simulink library "AEMS_Standard_Library"  (R2016b)
(part 4 of 39)

      |             end
      |         end
      |     end
      | 
      | %% Delete all AEMS_FLOAT_TO_FXP_WITH_LIMIT and AEMS_EXTRACT_BIT blocks
      |     k2=[find_system(hh,'FollowLinks','on','LookunderMasks','all','regexp','on','Name','^AEMS_TO_FXP_WITH_LIMIT');find_system(hh,'FollowLinks','on','LookunderMasks','all','MaskType','AEMS_EXTRACT_BIT')];
      | % if size(k,1)~= str2num(buf)
      |     for j = 1:length(k2)
      |         try
      |             delete_block(k2{j});
      |         end
      |     end
      | 
      | %% Settings for the Mux
      | % Number of inputs
      |     set_param([hh '/Mux'],'Inputs',num2str(buff_size));
      | 
      | % Mux position
      |     Blk.Position=get_param([hh '/Mux'],'position');
      |     Position = Blk.Position;
      |     Position(2) = pos(2) - 60*buff_size;
      |     Position(4) = pos(2) + 60*buff_size;
      |     set_param([hh '/Mux'],'Position', Position);
      |     inblkhandles=get_param([hh '/Mux'], 'PortHandles');
      | 
      |     set_param(hh,'Position',conv_sub_pos);
      | %% For each DID, recreate it
      |     i=0;
      |     txtvisibility='%<MaskType> \n DID Abstract: %<DIDAbstract> \n Number of DID Variables: %<NumDIDVar> ';
      |     for k=1:countDID
      |         k_str = num2str(k);
      | 
      |       try
      |         %% Add the DID information into the displayed text under the main lib block
      |         txtvisibility=[txtvisibility,'\n %<In_DID_Name_',k_str,'> : {','Range = %<RaDIDVar',k_str,'>, Resol = %<ResolDIDVar',k_str,'>, Offset = %<OffsetDIDVar',k_str,'>, DID Data Type= %<DataTypeDIDVar',k_str,'>}'];
      |         
      |         %% Retrieve all data from the DID tab  
      |         tRange = strsplit(strrep(strrep(strrep(get_param(libcb,['RaDIDVar',k_str]),' ',''),'[',''),']',''),',');
      |         tMin = tRange{1};
      |         tMax = tRange{2}; 
      |         tResol = get_param(libcb,['ResolDIDVar',k_str]);
      |         tOffset = get_param(libcb,['OffsetDIDVar',k_str]);
      |         
      |         tByte = get_param(libcb,['DataTypeDIDVar',k_str]);
      |         if(strcmp(tByte, 'int8') || strcmp (tByte, 'uint8'))
      |             t_buff_size=1;
      |         elseif(strcmp(tByte, 'int16') || strcmp (tByte, 'uint16'))
      |             t_buff_size=2;
      |         else
      |             t_buff_size=4;
      |         end
      |         
      | %% For each element in the buffer
      |         for ii=1:t_buff_size
      |             i=i+1;
      |             i_str = num2str(i);
      |             pos=get_param(inblkhandles.Inport(i),'position');
      |             cur_ext_bit = [hh '/AEMS_EXTRACT_BIT_',i_str];
      | 
      | %% Adding AEMS_EXTRACT_BIT if buffer > 1
      | % Adding block 
      |             if t_buff_size >= 1
      |                 add_block('AEMS_Standard_Library/BIT_OPERATION/AEMS_EXTRACT_BIT',cur_ext_bit,'Position',[pos(1)-300 pos(2)-15 pos(1)-100 pos(2)+15]);
      |                 %                     add_block('AEMS_Standard_Library/BIT_OPERATION/AEMS_EXTRACT_BIT',[hh '/AEMS_EXTRACT_BIT_' num2str(i)],'Position',[pos(1)-320 pos(2)-25 pos(1)-140 pos(2)+25]);
      |                 set_param(cur_ext_bit,'Value','Range of bits');
      |                 set_param(cur_ext_bit,'DataType',tByte);
      |             end
      |             
      | %% For the first byte in the buffer only, we create the input and float and fxp
      |             if ii==1
      |                 name_inpo = get_param(libcb,['In_DID_Name_',k_str]);
      |                 try
      |                     add_block('built-in/Inport',[hh '/DID_Variable_',k_str],'Position',[140 pos(2)-6 160 pos(2)+6],'BackGroundColor','Green');
      |                 catch
      |                   set_param([hh '/DID_Variable_',k_str],'Position',[140 pos(2)-6 160 pos(2)+6]);
      |                 end
      |                 
      | %% Add DataTypeConversion or AEMS_FLOAT_TO_FXP_WITH_LIMIT, and name them AEMS_FLOAT_TO_FXP_WITH_LIMIT_XX
      | % Remark Etienne: Not sure this part is right. User expects his data to be maxed at 1 in this case.               
      |                 flag_convert = 0;
      |                 try
      |                     if isequal({tResol,tMin,tMax,tOffset,tByte},{'1','0','1','0','1'})
      |                         add_block('built-in/DataTypeConversion',[hh '/AEMS_TO_FXP_WITH_LIMIT_',k_str],'Position',[pos(1)-620 pos(2)-20 pos(1)-555 pos(2)+15],'ShowName','off');
      |                         flag_convert = 1;
      |                     else
      |                         add_block('AEMS_Standard_Library/DCM/AEMS_TO_FXP_WITH_LIMIT',[hh '/AEMS_TO_FXP_WITH_LIMIT_',k_str],'Position',[pos(1)-720 pos(2)-20 pos(1)-460 pos(2)+20]);
      |                         set_param([hh '/AEMS_TO_FXP_WITH_LIMIT_',k_str],'OutputFixedPointDatatype',tByte);%Data type has to be set first before setting other attributes.                        
      |                         set_param([hh '/AEMS_TO_FXP_WITH_LIMIT_',k_str],...
      |                             'Resol',tResol,...
      |                             'Min',tMin,...
      |                             'Max',tMax,...
      |                             'Offset',tOffset);
      |                     end
      |                 end
      |                 
      | %% Setting lines and adding the inport
      |                 inp_k_pos = [40 conv_sub_pos(2)+10 60 conv_sub_pos(2)+22];
      |                 try
      |                     %                             add_line(hh,[name_inpo,'/1'],['AEMS_TO_FXP_WITH_LIMIT_',k_str,'/1'],'Autorouting','On');
      |                     
      |                     add_line(hh,['DID_Variable_',k_str,'/1'],['AEMS_TO_FXP_WITH_LIMIT_',k_str,'/1'],'Autorouting','On');
      |                     %                         add_block('built-in/Inport',[libcb '/DID_Variable_' num2str(k)],'Position',[posport(1)-10 posport(2)-6+k*100 posport(1)+10 posport(2)+6+k*100],'BackGroundColor','Green');
      |                     add_block('built-in/Inport',[libcb,'/DID_Variable_',k_str],'Position',inp_k_pos,'BackGroundColor','Green');
      |                     add_line(libcb,['DID_Variable_',k_str,'/1'],['Conversion_Subsystem/',k_str],'Autorouting','On');
      |                 catch
      |                     %                                                     set_param([libcb '/DID_Variable_' num2str(k)],'Position',[posport(1)-10 posport(2)-6+k*100 posport(1)+10 posport(2)+6+k*100]);
      |                     set_param([libcb,'/DID_Variable_',k_str],'Position',inp_k_pos);
      |                 end
      |             end
      |             
      |  %% Setting the range of bits to extract
      |             Start_Bit = (t_buff_size-ii)*8;
      |             End_Bit   = Start_Bit + 7;
      |             Range_Of_Bits = ['[',num2str(Start_Bit),',',num2str(End_Bit),']'];
      |             set_param(cur_ext_bit,'Range',Range_Of_Bits);
      |             
      | %% Linking the AEMS_FLOAT_TO_FXP_WITH_LIMIT and AEMS_EXTRACT_BIT_
      |             if t_buff_size > 0
      |                 add_line(hh,['AEMS_TO_FXP_WITH_LIMIT_',k_str,'/1'],['AEMS_EXTRACT_BIT_' num2str(i),'/1'], 'Autorouting','On');
      |                 add_line(hh,['AEMS_EXTRACT_BIT_',i_str,'/1'],['Mux/',i_str], 'Autorouting','On');
      |             end
      |         end
      |         
      |     catch error
      |         disp(error.message);
      |     end
      | end
      | 
      | %% Linking the inport for the Conversion_Subsystem
      |     ph_hh = get_param(hh,'PortHandles');
      |     ph_hh_in = ph_hh.Inport;
      |     for k1 = 1:countDID
      |         k1_str = num2str(k1);
      |         ph_hh_in_pos = get(ph_hh_in(k1),'Position');
      |         inp_k_pos = [40 ph_hh_in_pos(2)-6 60 ph_hh_in_pos(2)+6];
      |         set_param([libcb,'/DID_Variable_',k1_str],'Position',inp_k_pos);
      |         %             set_param([libcb,'/',name_inp1],'Position',inp_k_pos);
      |         try
      |             delete_line(libcb,['DID_Variable_',k1_str,'/1'],['Conversion_Subsystem/',k1_str]);
      |         catch
      |             disp('sf');
      |         end
      |         add_line(libcb,['DID_Variable_',k1_str,'/1'],['Conversion_Subsystem/',k1_str],'Autorouting','On');
      |     end
      |     
      | %% Setting position of the block relatively to the number of inputs
      |     prs_pos = get_param(libcb,'Position');
      |     if countDID > 4
      |         set_param(libcb,'Position',[prs_pos(1) prs_pos(2) prs_pos(3) prs_pos(2)+(countDID*30)]);
      |     else
      |         set_param(libcb,'Position',[prs_pos(1) prs_pos(2) prs_pos(3) prs_pos(2)+120]);
      |     end
      |     set_param(libcb,'AttributesFormatString',txtvisibility);
      | end
      | %% Setting the name of the DID in the inports
      |     fin_ip = find_system(libh,'LookUnderMasks','all','FollowLinks','on','SearchDepth','1','BlockType','Inport');
      |     for ip_cnt=1:length(fin_ip)
      |      cur_ip_name = get_param(libcb,['In_DID_Name_',num2str(ip_cnt)]);
      |         if ~isnan(str2double(cur_ip_name)) && isnumeric(str2double(cur_ip_name))
      |          errordlg(['invalid inport name entered for DID variable',num2str(ip_cnt)]);
      |         elseif ~isempty(cur_ip_name)
      |         try
      |             set(fin_ip(ip_cnt),'Name',cur_ip_name);
      |         catch
      |             errordlg(['invalid/duplicate inport name entered for DID variable',num2str(ip_cnt)]);
      |         end
      |         end
      |     end
      settings: AttributesFormatString=%<MaskType> \n DID Abstract: %<DIDAbstract> \n Number of DID Variables: %<NumDIDVar> \n %<In_DID_Name_1> : {Range = %<RaDIDVar1>, Resol = %<ResolDIDVar1>, Offset = %<OffsetDIDVar1>, DID Data Type= %<DataTypeDIDVar1>}
      mask Help:
      | eval('path_lib=fileparts(which(''AEMS_Standard_Library''));');
      | doc_path = [path_lib '\help\AEMS_DCM_DID_READDATA.pdf'];
      | eval('open(doc_path)')
      mask TypeOptions NumDIDVar: 1 | 2 | 3 | 4 | 5 | 6 | 7 | 8 | 9 | 10 | 11 | 12 | 13 | 14 | 15 | 16 | 17 | 18 | 19 | 20 | 21 | 22 | 23 | 24 | 25 | 26 | 27 | 28 | 29 | 30 | 31 | 32 | 33 | 34 | 35 | 36 | 37 | 38 | 39 | 40 | 41 | 42 | 43 | 44 | 45 | 46 | 47 | 48 | 49 | 50 | 51 | 52 | 53 | 54 | 55 | 56 | 57 | 58 | 59 | 60 | 61 | 62 | 63 | 64 | 65 | 66 | 67 | 68 | 69 | 70 | 71 | 72 | 73 | 74 | 75 | 76 | 77 | 78 | 79 | 80 | 81 | 82 | 83 | 84 | 85 | 86 | 87 | 88 | 89 | 90 | 91 | 92 | 93 | 94 | 95 | 96 | 97 | 98 | 99 | 100 | 101 | 102 | 103 | 104 | 105 | 106 | 107 | 108 | 109 | 110 | 111 | 112 | 113 | 114 | 115 | 116 | 117 | 118 | 119 | 120 | 121 | 122 | 123 | 124 | 125 | 126 | 127 | 128 | 129 | 130 | 131 | 132 | 133 | 134 | 135 | 136 | 137 | 138 | 139 | 140 | 141 | 142 | 143 | 144 | 145 | 146 | 147 | 148 | 149 | 150 | 151 | 152 | 153 | 154 | 155 | 156 | 157 | 158 | 159 | 160 | 161 | 162 | 163 | 164 | 165 | 166 | 167 | 168 | 169 | 170 | 171 | 172 | 173 | 174 | 175 | 176 | 177 | 178 | 179 | 180 | 181 | 182 | 183 | 184 | 185 | 186 | 187 | 188 | 189 | 190 | 191 | 192 | 193 | 194 | 195 | 196 | 197 | 198 | 199 | 200 | 201 | 202 | 203 | 204 | 205 | 206 | 207 | 208 | 209 | 210 | 211 | 212 | 213 | 214 | 215 | 216 | 217 | 218 | 219 | 220 | 221 | 222 | 223 | 224 | 225 | 226 | 227 | 228 | 229 | 230 | 231 | 232 | 233 | 234 | 235 | 236 | 237 | 238 | 239 | 240 | 241 | 242 | 243 | 244 | 245 | 246 | 247 | 248 | 249 | 250 | 251 | 252 | 253 | 254 | 255 | 256 | 257 | 258 | 259 | 260 | 261 | 262 | 263 | 264 | 265 | 266 | 267 | 268 | 269 | 270 | 271 | 272 | 273 | 274 | 275 | 276 | 277 | 278 | 279 | 280 | 281 | 282 | 283 | 284 | 285 | 286 | 287 | 288 | 289 | 290 | 291 | 292 | 293 | 294 | 295 | 296 | 297 | 298 | 299 | 300 | 301 | 302 | 303 | 304 | 305 | 306 | 307 | 308 | 309 | 310 | 311 | 312 | 313 | 314 | 315 | 316 | 317 | 318 | 319 | 320 | 321 | 322 | 323 | 324 | 325 | 326 | 327 | 328 | 329 | 330 | 331 | 332 | 333 | 334 | 335 | 336 | 337 | 338 | 339 | 340 | 341 | 342 | 343 | 344 | 345 | 346 | 347 | 348 | 349 | 350 | 351 | 352 | 353 | 354 | 355 | 356 | 357 | 358 | 359 | 360 | 361 | 362 | 363 | 364 | 365 | 366 | 367 | 368 | 369 | 370 | 371 | 372 | 373 | 374 | 375 | 376 | 377 | 378 | 379 | 380 | 381 | 382 | 383 | 384 | 385 | 386 | 387 | 388 | 389 | 390 | 391 | 392 | 393 | 394 | 395 | 396 | 397 | 398 | 399 | 400
      mask Callback NumDIDVar:
      | mo = get_param(gcb,'MaskObject');
      | %Get number of tabs in container 2
      | NumOfTabs = mo.getDialogControl('tabgroup');
      | % Set visibility off from 2
      | for i = 2:length(NumOfTabs.DialogControls)
      |     NumOfTabs.DialogControls(i).Visible ='off';
      | end
      | 
      | Value = str2double(get(gcbh,'NumDIDVar'));
      | 
      | for s = 2:Value+1
      |     NumOfTabs.DialogControls(s).Visible ='on';
      | end
      mask TypeOptions DataTypeDIDVar1: uint8 | int8 | uint16 | int16 | uint32 | int32
      mask TypeOptions DataTypeDIDVar2: uint8 | int8 | uint16 | int16 | uint32 | int32
      mask TypeOptions DataTypeDIDVar3: uint8 | int8 | uint16 | int16 | uint32 | int32
      mask TypeOptions DataTypeDIDVar4: uint8 | int8 | uint16 | int16 | uint32 | int32
      mask TypeOptions DataTypeDIDVar5: uint8 | int8 | uint16 | int16 | uint32 | int32
      mask TypeOptions DataTypeDIDVar6: uint8 | int8 | uint16 | int16 | uint32 | int32
      mask TypeOptions DataTypeDIDVar7: uint8 | int8 | uint16 | int16 | uint32 | int32
      mask TypeOptions DataTypeDIDVar8: uint8 | int8 | uint16 | int16 | uint32 | int32
      mask TypeOptions DataTypeDIDVar9: uint8 | int8 | uint16 | int16 | uint32 | int32
      mask TypeOptions DataTypeDIDVar10: uint8 | int8 | uint16 | int16 | uint32 | int32
      mask TypeOptions DataTypeDIDVar11: uint8 | int8 | uint16 | int16 | uint32 | int32
      mask TypeOptions DataTypeDIDVar12: uint8 | int8 | uint16 | int16 | uint32 | int32
      mask TypeOptions DataTypeDIDVar13: uint8 | int8 | uint16 | int16 | uint32 | int32
      mask TypeOptions DataTypeDIDVar14: uint8 | int8 | uint16 | int16 | uint32 | int32
      mask TypeOptions DataTypeDIDVar15: uint8 | int8 | uint16 | int16 | uint32 | int32
      mask TypeOptions DataTypeDIDVar16: uint8 | int8 | uint16 | int16 | uint32 | int32
      mask TypeOptions DataTypeDIDVar17: uint8 | int8 | uint16 | int16 | uint32 | int32
      mask TypeOptions DataTypeDIDVar18: uint8 | int8 | uint16 | int16 | uint32 | int32
      mask TypeOptions DataTypeDIDVar19: uint8 | int8 | uint16 | int16 | uint32 | int32
      mask TypeOptions DataTypeDIDVar20: uint8 | int8 | uint16 | int16 | uint32 | int32
      mask TypeOptions DataTypeDIDVar21: uint8 | int8 | uint16 | int16 | uint32 | int32
      mask TypeOptions DataTypeDIDVar22: uint8 | int8 | uint16 | int16 | uint32 | int32
      mask TypeOptions DataTypeDIDVar23: uint8 | int8 | uint16 | int16 | uint32 | int32
      mask TypeOptions DataTypeDIDVar24: uint8 | int8 | uint16 | int16 | uint32 | int32
      mask TypeOptions DataTypeDIDVar25: uint8 | int8 | uint16 | int16 | uint32 | int32
      mask TypeOptions DataTypeDIDVar26: uint8 | int8 | uint16 | int16 | uint32 | int32
      mask TypeOptions DataTypeDIDVar27: uint8 | int8 | uint16 | int16 | uint32 | int32
      mask TypeOptions DataTypeDIDVar28: uint8 | int8 | uint16 | int16 | uint32 | int32
      mask TypeOptions DataTypeDIDVar29: uint8 | int8 | uint16 | int16 | uint32 | int32
      mask TypeOptions DataTypeDIDVar30: uint8 | int8 | uint16 | int16 | uint32 | int32
      mask TypeOptions DataTypeDIDVar31: uint8 | int8 | uint16 | int16 | uint32 | int32
      mask TypeOptions DataTypeDIDVar32: uint8 | int8 | uint16 | int16 | uint32 | int32
      mask TypeOptions DataTypeDIDVar33: uint8 | int8 | uint16 | int16 | uint32 | int32
      mask TypeOptions DataTypeDIDVar34: uint8 | int8 | uint16 | int16 | uint32 | int32
      mask TypeOptions DataTypeDIDVar35: uint8 | int8 | uint16 | int16 | uint32 | int32
      mask TypeOptions DataTypeDIDVar36: uint8 | int8 | uint16 | int16 | uint32 | int32
      mask TypeOptions DataTypeDIDVar37: uint8 | int8 | uint16 | int16 | uint32 | int32
      mask TypeOptions DataTypeDIDVar38: uint8 | int8 | uint16 | int16 | uint32 | int32
      mask TypeOptions DataTypeDIDVar39: uint8 | int8 | uint16 | int16 | uint32 | int32
      mask TypeOptions DataTypeDIDVar40: uint8 | int8 | uint16 | int16 | uint32 | int32
      mask TypeOptions DataTypeDIDVar41: uint8 | int8 | uint16 | int16 | uint32 | int32
      mask TypeOptions DataTypeDIDVar42: uint8 | int8 | uint16 | int16 | uint32 | int32
      mask TypeOptions DataTypeDIDVar43: uint8 | int8 | uint16 | int16 | uint32 | int32
      mask TypeOptions DataTypeDIDVar44: uint8 | int8 | uint16 | int16 | uint32 | int32
      mask TypeOptions DataTypeDIDVar45: uint8 | int8 | uint16 | int16 | uint32 | int32
      mask TypeOptions DataTypeDIDVar46: uint8 | int8 | uint16 | int16 | uint32 | int32
      mask TypeOptions DataTypeDIDVar47: uint8 | int8 | uint16 | int16 | uint32 | int32
      mask TypeOptions DataTypeDIDVar48: uint8 | int8 | uint16 | int16 | uint32 | int32
      mask TypeOptions DataTypeDIDVar49: uint8 | int8 | uint16 | int16 | uint32 | int32
      mask TypeOptions DataTypeDIDVar50: uint8 | int8 | uint16 | int16 | uint32 | int32
      mask TypeOptions DataTypeDIDVar51: uint8 | int8 | uint16 | int16 | uint32 | int32
      mask TypeOptions DataTypeDIDVar52: uint8 | int8 | uint16 | int16 | uint32 | int32
      mask TypeOptions DataTypeDIDVar53: uint8 | int8 | uint16 | int16 | uint32 | int32
      mask TypeOptions DataTypeDIDVar54: uint8 | int8 | uint16 | int16 | uint32 | int32
      mask TypeOptions DataTypeDIDVar55: uint8 | int8 | uint16 | int16 | uint32 | int32
      mask TypeOptions DataTypeDIDVar56: uint8 | int8 | uint16 | int16 | uint32 | int32
      mask TypeOptions DataTypeDIDVar57: uint8 | int8 | uint16 | int16 | uint32 | int32
      mask TypeOptions DataTypeDIDVar58: uint8 | int8 | uint16 | int16 | uint32 | int32
      mask TypeOptions DataTypeDIDVar59: uint8 | int8 | uint16 | int16 | uint32 | int32
      mask TypeOptions DataTypeDIDVar60: uint8 | int8 | uint16 | int16 | uint32 | int32
      mask TypeOptions DataTypeDIDVar61: uint8 | int8 | uint16 | int16 | uint32 | int32
      mask TypeOptions DataTypeDIDVar62: uint8 | int8 | uint16 | int16 | uint32 | int32
      mask TypeOptions DataTypeDIDVar63: uint8 | int8 | uint16 | int16 | uint32 | int32
      mask TypeOptions DataTypeDIDVar64: uint8 | int8 | uint16 | int16 | uint32 | int32
      mask TypeOptions DataTypeDIDVar65: uint8 | int8 | uint16 | int16 | uint32 | int32
      mask TypeOptions DataTypeDIDVar66: uint8 | int8 | uint16 | int16 | uint32 | int32
      mask TypeOptions DataTypeDIDVar67: uint8 | int8 | uint16 | int16 | uint32 | int32
      mask TypeOptions DataTypeDIDVar68: uint8 | int8 | uint16 | int16 | uint32 | int32
      mask TypeOptions DataTypeDIDVar69: uint8 | int8 | uint16 | int16 | uint32 | int32
      mask TypeOptions DataTypeDIDVar70: uint8 | int8 | uint16 | int16 | uint32 | int32
      mask TypeOptions DataTypeDIDVar71: uint8 | int8 | uint16 | int16 | uint32 | int32
      mask TypeOptions DataTypeDIDVar72: uint8 | int8 | uint16 | int16 | uint32 | int32
      mask TypeOptions DataTypeDIDVar73: uint8 | int8 | uint16 | int16 | uint32 | int32
      mask TypeOptions DataTypeDIDVar74: uint8 | int8 | uint16 | int16 | uint32 | int32
      mask TypeOptions DataTypeDIDVar75: uint8 | int8 | uint16 | int16 | uint32 | int32
      mask TypeOptions DataTypeDIDVar76: uint8 | int8 | uint16 | int16 | uint32 | int32
      mask TypeOptions DataTypeDIDVar77: uint8 | int8 | uint16 | int16 | uint32 | int32
      mask TypeOptions DataTypeDIDVar78: uint8 | int8 | uint16 | int16 | uint32 | int32
      mask TypeOptions DataTypeDIDVar79: uint8 | int8 | uint16 | int16 | uint32 | int32
      mask TypeOptions DataTypeDIDVar80: uint8 | int8 | uint16 | int16 | uint32 | int32
      mask TypeOptions DataTypeDIDVar81: uint8 | int8 | uint16 | int16 | uint32 | int32
      mask TypeOptions DataTypeDIDVar82: uint8 | int8 | uint16 | int16 | uint32 | int32
      mask TypeOptions DataTypeDIDVar83: uint8 | int8 | uint16 | int16 | uint32 | int32
      mask TypeOptions DataTypeDIDVar84: uint8 | int8 | uint16 | int16 | uint32 | int32
      mask TypeOptions DataTypeDIDVar85: uint8 | int8 | uint16 | int16 | uint32 | int32
      mask TypeOptions DataTypeDIDVar86: uint8 | int8 | uint16 | int16 | uint32 | int32
      mask TypeOptions DataTypeDIDVar87: uint8 | int8 | uint16 | int16 | uint32 | int32
      mask TypeOptions DataTypeDIDVar88: uint8 | int8 | uint16 | int16 | uint32 | int32
      mask TypeOptions DataTypeDIDVar89: uint8 | int8 | uint16 | int16 | uint32 | int32
      mask TypeOptions DataTypeDIDVar90: uint8 | int8 | uint16 | int16 | uint32 | int32
      mask TypeOptions DataTypeDIDVar91: uint8 | int8 | uint16 | int16 | uint32 | int32
      mask TypeOptions DataTypeDIDVar92: uint8 | int8 | uint16 | int16 | uint32 | int32
      mask TypeOptions DataTypeDIDVar93: uint8 | int8 | uint16 | int16 | uint32 | int32
      mask TypeOptions DataTypeDIDVar94: uint8 | int8 | uint16 | int16 | uint32 | int32
      mask TypeOptions DataTypeDIDVar95: uint8 | int8 | uint16 | int16 | uint32 | int32
      mask TypeOptions DataTypeDIDVar96: uint8 | int8 | uint16 | int16 | uint32 | int32
      mask TypeOptions DataTypeDIDVar97: uint8 | int8 | uint16 | int16 | uint32 | int32
      mask TypeOptions DataTypeDIDVar98: uint8 | int8 | uint16 | int16 | uint32 | int32
      mask TypeOptions DataTypeDIDVar99: uint8 | int8 | uint16 | int16 | uint32 | int32
      mask TypeOptions DataTypeDIDVar100: uint8 | int8 | uint16 | int16 | uint32 | int32
      mask TypeOptions DataTypeDIDVar101: uint8 | int8 | uint16 | int16 | uint32 | int32
      mask TypeOptions DataTypeDIDVar102: uint8 | int8 | uint16 | int16 | uint32 | int32
      mask TypeOptions DataTypeDIDVar103: uint8 | int8 | uint16 | int16 | uint32 | int32
      mask TypeOptions DataTypeDIDVar104: uint8 | int8 | uint16 | int16 | uint32 | int32
      mask TypeOptions DataTypeDIDVar105: uint8 | int8 | uint16 | int16 | uint32 | int32
      mask TypeOptions DataTypeDIDVar106: uint8 | int8 | uint16 | int16 | uint32 | int32
      mask TypeOptions DataTypeDIDVar107: uint8 | int8 | uint16 | int16 | uint32 | int32
      mask TypeOptions DataTypeDIDVar108: uint8 | int8 | uint16 | int16 | uint32 | int32
      mask TypeOptions DataTypeDIDVar109: uint8 | int8 | uint16 | int16 | uint32 | int32
      mask TypeOptions DataTypeDIDVar110: uint8 | int8 | uint16 | int16 | uint32 | int32
      mask TypeOptions DataTypeDIDVar111: uint8 | int8 | uint16 | int16 | uint32 | int32
      mask TypeOptions DataTypeDIDVar112: uint8 | int8 | uint16 | int16 | uint32 | int32
      mask TypeOptions DataTypeDIDVar113: uint8 | int8 | uint16 | int16 | uint32 | int32
      mask TypeOptions DataTypeDIDVar114: uint8 | int8 | uint16 | int16 | uint32 | int32
      mask TypeOptions DataTypeDIDVar115: uint8 | int8 | uint16 | int16 | uint32 | int32
      mask TypeOptions DataTypeDIDVar116: uint8 | int8 | uint16 | int16 | uint32 | int32
      mask TypeOptions DataTypeDIDVar117: uint8 | int8 | uint16 | int16 | uint32 | int32
      mask TypeOptions DataTypeDIDVar118: uint8 | int8 | uint16 | int16 | uint32 | int32
      mask TypeOptions DataTypeDIDVar119: uint8 | int8 | uint16 | int16 | uint32 | int32
      mask TypeOptions DataTypeDIDVar120: uint8 | int8 | uint16 | int16 | uint32 | int32
      mask TypeOptions DataTypeDIDVar121: uint8 | int8 | uint16 | int16 | uint32 | int32
      mask TypeOptions DataTypeDIDVar122: uint8 | int8 | uint16 | int16 | uint32 | int32
      mask TypeOptions DataTypeDIDVar123: uint8 | int8 | uint16 | int16 | uint32 | int32
      mask TypeOptions DataTypeDIDVar124: uint8 | int8 | uint16 | int16 | uint32 | int32
      mask TypeOptions DataTypeDIDVar125: uint8 | int8 | uint16 | int16 | uint32 | int32
      mask TypeOptions DataTypeDIDVar126: uint8 | int8 | uint16 | int16 | uint32 | int32
      mask TypeOptions DataTypeDIDVar127: uint8 | int8 | uint16 | int16 | uint32 | int32
      mask TypeOptions DataTypeDIDVar128: uint8 | int8 | uint16 | int16 | uint32 | int32
      mask TypeOptions DataTypeDIDVar129: uint8 | int8 | uint16 | int16 | uint32 | int32
      mask TypeOptions DataTypeDIDVar130: uint8 | int8 | uint16 | int16 | uint32 | int32
      mask TypeOptions DataTypeDIDVar131: uint8 | int8 | uint16 | int16 | uint32 | int32
      mask TypeOptions DataTypeDIDVar132: uint8 | int8 | uint16 | int16 | uint32 | int32
      mask TypeOptions DataTypeDIDVar133: uint8 | int8 | uint16 | int16 | uint32 | int32
      mask TypeOptions DataTypeDIDVar134: uint8 | int8 | uint16 | int16 | uint32 | int32
      mask TypeOptions DataTypeDIDVar135: uint8 | int8 | uint16 | int16 | uint32 | int32
      mask TypeOptions DataTypeDIDVar136: uint8 | int8 | uint16 | int16 | uint32 | int32
      mask TypeOptions DataTypeDIDVar137: uint8 | int8 | uint16 | int16 | uint32 | int32
      mask TypeOptions DataTypeDIDVar138: uint8 | int8 | uint16 | int16 | uint32 | int32
      mask TypeOptions DataTypeDIDVar139: uint8 | int8 | uint16 | int16 | uint32 | int32
      mask TypeOptions DataTypeDIDVar140: uint8 | int8 | uint16 | int16 | uint32 | int32
      mask TypeOptions DataTypeDIDVar141: uint8 | int8 | uint16 | int16 | uint32 | int32
      mask TypeOptions DataTypeDIDVar142: uint8 | int8 | uint16 | int16 | uint32 | int32
      mask TypeOptions DataTypeDIDVar143: uint8 | int8 | uint16 | int16 | uint32 | int32
      mask TypeOptions DataTypeDIDVar144: uint8 | int8 | uint16 | int16 | uint32 | int32
      mask TypeOptions DataTypeDIDVar145: uint8 | int8 | uint16 | int16 | uint32 | int32
      mask TypeOptions DataTypeDIDVar146: uint8 | int8 | uint16 | int16 | uint32 | int32
      mask TypeOptions DataTypeDIDVar147: uint8 | int8 | uint16 | int16 | uint32 | int32
      mask TypeOptions DataTypeDIDVar148: uint8 | int8 | uint16 | int16 | uint32 | int32
      mask TypeOptions DataTypeDIDVar149: uint8 | int8 | uint16 | int16 | uint32 | int32
      mask TypeOptions DataTypeDIDVar150: uint8 | int8 | uint16 | int16 | uint32 | int32
      mask TypeOptions DataTypeDIDVar151: uint8 | int8 | uint16 | int16 | uint32 | int32
      mask TypeOptions DataTypeDIDVar152: uint8 | int8 | uint16 | int16 | uint32 | int32
      mask TypeOptions DataTypeDIDVar153: uint8 | int8 | uint16 | int16 | uint32 | int32
      mask TypeOptions DataTypeDIDVar154: uint8 | int8 | uint16 | int16 | uint32 | int32
      mask TypeOptions DataTypeDIDVar155: uint8 | int8 | uint16 | int16 | uint32 | int32
      mask TypeOptions DataTypeDIDVar156: uint8 | int8 | uint16 | int16 | uint32 | int32
      mask TypeOptions DataTypeDIDVar157: uint8 | int8 | uint16 | int16 | uint32 | int32
      mask TypeOptions DataTypeDIDVar158: uint8 | int8 | uint16 | int16 | uint32 | int32
      mask TypeOptions DataTypeDIDVar159: uint8 | int8 | uint16 | int16 | uint32 | int32
      mask TypeOptions DataTypeDIDVar160: uint8 | int8 | uint16 | int16 | uint32 | int32
      mask TypeOptions DataTypeDIDVar161: uint8 | int8 | uint16 | int16 | uint32 | int32
      mask TypeOptions DataTypeDIDVar162: uint8 | int8 | uint16 | int16 | uint32 | int32
      mask TypeOptions DataTypeDIDVar163: uint8 | int8 | uint16 | int16 | uint32 | int32
      mask TypeOptions DataTypeDIDVar164: uint8 | int8 | uint16 | int16 | uint32 | int32
      mask TypeOptions DataTypeDIDVar165: uint8 | int8 | uint16 | int16 | uint32 | int32
      mask TypeOptions DataTypeDIDVar166: uint8 | int8 | uint16 | int16 | uint32 | int32
      mask TypeOptions DataTypeDIDVar167: uint8 | int8 | uint16 | int16 | uint32 | int32
      mask TypeOptions DataTypeDIDVar168: uint8 | int8 | uint16 | int16 | uint32 | int32
      mask TypeOptions DataTypeDIDVar169: uint8 | int8 | uint16 | int16 | uint32 | int32
      mask TypeOptions DataTypeDIDVar170: uint8 | int8 | uint16 | int16 | uint32 | int32
      mask TypeOptions DataTypeDIDVar171: uint8 | int8 | uint16 | int16 | uint32 | int32
      mask TypeOptions DataTypeDIDVar172: uint8 | int8 | uint16 | int16 | uint32 | int32
      mask TypeOptions DataTypeDIDVar173: uint8 | int8 | uint16 | int16 | uint32 | int32
      mask TypeOptions DataTypeDIDVar174: uint8 | int8 | uint16 | int16 | uint32 | int32
      mask TypeOptions DataTypeDIDVar175: uint8 | int8 | uint16 | int16 | uint32 | int32
      mask TypeOptions DataTypeDIDVar176: uint8 | int8 | uint16 | int16 | uint32 | int32
      mask TypeOptions DataTypeDIDVar177: uint8 | int8 | uint16 | int16 | uint32 | int32
      mask TypeOptions DataTypeDIDVar178: uint8 | int8 | uint16 | int16 | uint32 | int32
      mask TypeOptions DataTypeDIDVar179: uint8 | int8 | uint16 | int16 | uint32 | int32
      mask TypeOptions DataTypeDIDVar180: uint8 | int8 | uint16 | int16 | uint32 | int32
      mask TypeOptions DataTypeDIDVar181: uint8 | int8 | uint16 | int16 | uint32 | int32
      mask TypeOptions DataTypeDIDVar182: uint8 | int8 | uint16 | int16 | uint32 | int32
      mask TypeOptions DataTypeDIDVar183: uint8 | int8 | uint16 | int16 | uint32 | int32
      mask TypeOptions DataTypeDIDVar184: uint8 | int8 | uint16 | int16 | uint32 | int32
      mask TypeOptions DataTypeDIDVar185: uint8 | int8 | uint16 | int16 | uint32 | int32
      mask TypeOptions DataTypeDIDVar186: uint8 | int8 | uint16 | int16 | uint32 | int32
      mask TypeOptions DataTypeDIDVar187: uint8 | int8 | uint16 | int16 | uint32 | int32
      mask TypeOptions DataTypeDIDVar188: uint8 | int8 | uint16 | int16 | uint32 | int32
      mask TypeOptions DataTypeDIDVar189: uint8 | int8 | uint16 | int16 | uint32 | int32
      mask TypeOptions DataTypeDIDVar190: uint8 | int8 | uint16 | int16 | uint32 | int32
      mask TypeOptions DataTypeDIDVar191: uint8 | int8 | uint16 | int16 | uint32 | int32
      mask TypeOptions DataTypeDIDVar192: uint8 | int8 | uint16 | int16 | uint32 | int32
      mask TypeOptions DataTypeDIDVar193: uint8 | int8 | uint16 | int16 | uint32 | int32
      mask TypeOptions DataTypeDIDVar194: uint8 | int8 | uint16 | int16 | uint32 | int32
      mask TypeOptions DataTypeDIDVar195: uint8 | int8 | uint16 | int16 | uint32 | int32
      mask TypeOptions DataTypeDIDVar196: uint8 | int8 | uint16 | int16 | uint32 | int32
      mask TypeOptions DataTypeDIDVar197: uint8 | int8 | uint16 | int16 | uint32 | int32
      mask TypeOptions DataTypeDIDVar198: uint8 | int8 | uint16 | int16 | uint32 | int32
      mask TypeOptions DataTypeDIDVar199: uint8 | int8 | uint16 | int16 | uint32 | int32
      mask TypeOptions DataTypeDIDVar200: uint8 | int8 | uint16 | int16 | uint32 | int32
      mask TypeOptions DataTypeDIDVar201: uint8 | int8 | uint16 | int16 | uint32 | int32
      mask TypeOptions DataTypeDIDVar202: uint8 | int8 | uint16 | int16 | uint32 | int32
      mask TypeOptions DataTypeDIDVar203: uint8 | int8 | uint16 | int16 | uint32 | int32
      mask TypeOptions DataTypeDIDVar204: uint8 | int8 | uint16 | int16 | uint32 | int32
      mask TypeOptions DataTypeDIDVar205: uint8 | int8 | uint16 | int16 | uint32 | int32
      mask TypeOptions DataTypeDIDVar206: uint8 | int8 | uint16 | int16 | uint32 | int32
      mask TypeOptions DataTypeDIDVar207: uint8 | int8 | uint16 | int16 | uint32 | int32
      mask TypeOptions DataTypeDIDVar208: uint8 | int8 | uint16 | int16 | uint32 | int32
      mask TypeOptions DataTypeDIDVar209: uint8 | int8 | uint16 | int16 | uint32 | int32
      mask TypeOptions DataTypeDIDVar210: uint8 | int8 | uint16 | int16 | uint32 | int32
      mask TypeOptions DataTypeDIDVar211: uint8 | int8 | uint16 | int16 | uint32 | int32
      mask TypeOptions DataTypeDIDVar212: uint8 | int8 | uint16 | int16 | uint32 | int32
      mask TypeOptions DataTypeDIDVar213: uint8 | int8 | uint16 | int16 | uint32 | int32
      mask TypeOptions DataTypeDIDVar214: uint8 | int8 | uint16 | int16 | uint32 | int32
      mask TypeOptions DataTypeDIDVar215: uint8 | int8 | uint16 | int16 | uint32 | int32
      mask TypeOptions DataTypeDIDVar216: uint8 | int8 | uint16 | int16 | uint32 | int32
      mask TypeOptions DataTypeDIDVar217: uint8 | int8 | uint16 | int16 | uint32 | int32
      mask TypeOptions DataTypeDIDVar218: uint8 | int8 | uint16 | int16 | uint32 | int32
      mask TypeOptions DataTypeDIDVar219: uint8 | int8 | uint16 | int16 | uint32 | int32
      mask TypeOptions DataTypeDIDVar220: uint8 | int8 | uint16 | int16 | uint32 | int32
      mask TypeOptions DataTypeDIDVar221: uint8 | int8 | uint16 | int16 | uint32 | int32
      mask TypeOptions DataTypeDIDVar222: uint8 | int8 | uint16 | int16 | uint32 | int32
      mask TypeOptions DataTypeDIDVar223: uint8 | int8 | uint16 | int16 | uint32 | int32
      mask TypeOptions DataTypeDIDVar224: uint8 | int8 | uint16 | int16 | uint32 | int32
      mask TypeOptions DataTypeDIDVar225: uint8 | int8 | uint16 | int16 | uint32 | int32
      mask TypeOptions DataTypeDIDVar226: uint8 | int8 | uint16 | int16 | uint32 | int32
      mask TypeOptions DataTypeDIDVar227: uint8 | int8 | uint16 | int16 | uint32 | int32
      mask TypeOptions DataTypeDIDVar228: uint8 | int8 | uint16 | int16 | uint32 | int32
      mask TypeOptions DataTypeDIDVar229: uint8 | int8 | uint16 | int16 | uint32 | int32
      mask TypeOptions DataTypeDIDVar230: uint8 | int8 | uint16 | int16 | uint32 | int32
      mask TypeOptions DataTypeDIDVar231: uint8 | int8 | uint16 | int16 | uint32 | int32
      mask TypeOptions DataTypeDIDVar232: uint8 | int8 | uint16 | int16 | uint32 | int32
      mask TypeOptions DataTypeDIDVar233: uint8 | int8 | uint16 | int16 | uint32 | int32
      mask TypeOptions DataTypeDIDVar234: uint8 | int8 | uint16 | int16 | uint32 | int32
      mask TypeOptions DataTypeDIDVar235: uint8 | int8 | uint16 | int16 | uint32 | int32
      mask TypeOptions DataTypeDIDVar236: uint8 | int8 | uint16 | int16 | uint32 | int32
      mask TypeOptions DataTypeDIDVar237: uint8 | int8 | uint16 | int16 | uint32 | int32
      mask TypeOptions DataTypeDIDVar238: uint8 | int8 | uint16 | int16 | uint32 | int32
      mask TypeOptions DataTypeDIDVar239: uint8 | int8 | uint16 | int16 | uint32 | int32
      mask TypeOptions DataTypeDIDVar240: uint8 | int8 | uint16 | int16 | uint32 | int32
      mask TypeOptions DataTypeDIDVar241: uint8 | int8 | uint16 | int16 | uint32 | int32
      mask TypeOptions DataTypeDIDVar242: uint8 | int8 | uint16 | int16 | uint32 | int32
      mask TypeOptions DataTypeDIDVar243: uint8 | int8 | uint16 | int16 | uint32 | int32
      mask TypeOptions DataTypeDIDVar244: uint8 | int8 | uint16 | int16 | uint32 | int32
      mask TypeOptions DataTypeDIDVar245: uint8 | int8 | uint16 | int16 | uint32 | int32
      mask TypeOptions DataTypeDIDVar246: uint8 | int8 | uint16 | int16 | uint32 | int32
      mask TypeOptions DataTypeDIDVar247: uint8 | int8 | uint16 | int16 | uint32 | int32
      mask TypeOptions DataTypeDIDVar248: uint8 | int8 | uint16 | int16 | uint32 | int32
      mask TypeOptions DataTypeDIDVar249: uint8 | int8 | uint16 | int16 | uint32 | int32
      mask TypeOptions DataTypeDIDVar250: uint8 | int8 | uint16 | int16 | uint32 | int32
      mask TypeOptions DataTypeDIDVar251: uint8 | int8 | uint16 | int16 | uint32 | int32
      mask TypeOptions DataTypeDIDVar252: uint8 | int8 | uint16 | int16 | uint32 | int32
      mask TypeOptions DataTypeDIDVar253: uint8 | int8 | uint16 | int16 | uint32 | int32
      mask TypeOptions DataTypeDIDVar254: uint8 | int8 | uint16 | int16 | uint32 | int32
      mask TypeOptions DataTypeDIDVar255: uint8 | int8 | uint16 | int16 | uint32 | int32
      mask TypeOptions DataTypeDIDVar256: uint8 | int8 | uint16 | int16 | uint32 | int32
      mask TypeOptions DataTypeDIDVar257: uint8 | int8 | uint16 | int16 | uint32 | int32
      mask TypeOptions DataTypeDIDVar258: uint8 | int8 | uint16 | int16 | uint32 | int32
      mask TypeOptions DataTypeDIDVar259: uint8 | int8 | uint16 | int16 | uint32 | int32
      mask TypeOptions DataTypeDIDVar260: uint8 | int8 | uint16 | int16 | uint32 | int32
      mask TypeOptions DataTypeDIDVar261: uint8 | int8 | uint16 | int16 | uint32 | int32
      mask TypeOptions DataTypeDIDVar262: uint8 | int8 | uint16 | int16 | uint32 | int32
      mask TypeOptions DataTypeDIDVar263: uint8 | int8 | uint16 | int16 | uint32 | int32
      mask TypeOptions DataTypeDIDVar264: uint8 | int8 | uint16 | int16 | uint32 | int32
      mask TypeOptions DataTypeDIDVar265: uint8 | int8 | uint16 | int16 | uint32 | int32
      mask TypeOptions DataTypeDIDVar266: uint8 | int8 | uint16 | int16 | uint32 | int32
      mask TypeOptions DataTypeDIDVar267: uint8 | int8 | uint16 | int16 | uint32 | int32
      mask TypeOptions DataTypeDIDVar268: uint8 | int8 | uint16 | int16 | uint32 | int32
      mask TypeOptions DataTypeDIDVar269: uint8 | int8 | uint16 | int16 | uint32 | int32
      mask TypeOptions DataTypeDIDVar270: uint8 | int8 | uint16 | int16 | uint32 | int32
      mask TypeOptions DataTypeDIDVar271: uint8 | int8 | uint16 | int16 | uint32 | int32
      mask TypeOptions DataTypeDIDVar272: uint8 | int8 | uint16 | int16 | uint32 | int32
      mask TypeOptions DataTypeDIDVar273: uint8 | int8 | uint16 | int16 | uint32 | int32
      mask TypeOptions DataTypeDIDVar274: uint8 | int8 | uint16 | int16 | uint32 | int32
      mask TypeOptions DataTypeDIDVar275: uint8 | int8 | uint16 | int16 | uint32 | int32
      mask TypeOptions DataTypeDIDVar276: uint8 | int8 | uint16 | int16 | uint32 | int32
      mask TypeOptions DataTypeDIDVar277: uint8 | int8 | uint16 | int16 | uint32 | int32
      mask TypeOptions DataTypeDIDVar278: uint8 | int8 | uint16 | int16 | uint32 | int32
      mask TypeOptions DataTypeDIDVar279: uint8 | int8 | uint16 | int16 | uint32 | int32
      mask TypeOptions DataTypeDIDVar280: uint8 | int8 | uint16 | int16 | uint32 | int32
      mask TypeOptions DataTypeDIDVar281: uint8 | int8 | uint16 | int16 | uint32 | int32
      mask TypeOptions DataTypeDIDVar282: uint8 | int8 | uint16 | int16 | uint32 | int32
      mask TypeOptions DataTypeDIDVar283: uint8 | int8 | uint16 | int16 | uint32 | int32
      mask TypeOptions DataTypeDIDVar284: uint8 | int8 | uint16 | int16 | uint32 | int32
      mask TypeOptions DataTypeDIDVar285: uint8 | int8 | uint16 | int16 | uint32 | int32
      mask TypeOptions DataTypeDIDVar286: uint8 | int8 | uint16 | int16 | uint32 | int32
      mask TypeOptions DataTypeDIDVar287: uint8 | int8 | uint16 | int16 | uint32 | int32
      mask TypeOptions DataTypeDIDVar288: uint8 | int8 | uint16 | int16 | uint32 | int32
      mask TypeOptions DataTypeDIDVar289: uint8 | int8 | uint16 | int16 | uint32 | int32
      mask TypeOptions DataTypeDIDVar290: uint8 | int8 | uint16 | int16 | uint32 | int32
      mask TypeOptions DataTypeDIDVar291: uint8 | int8 | uint16 | int16 | uint32 | int32
      mask TypeOptions DataTypeDIDVar292: uint8 | int8 | uint16 | int16 | uint32 | int32
      mask TypeOptions DataTypeDIDVar293: uint8 | int8 | uint16 | int16 | uint32 | int32
      mask TypeOptions DataTypeDIDVar294: uint8 | int8 | uint16 | int16 | uint32 | int32
      mask TypeOptions DataTypeDIDVar295: uint8 | int8 | uint16 | int16 | uint32 | int32
      mask TypeOptions DataTypeDIDVar296: uint8 | int8 | uint16 | int16 | uint32 | int32
      mask TypeOptions DataTypeDIDVar297: uint8 | int8 | uint16 | int16 | uint32 | int32
      mask TypeOptions DataTypeDIDVar298: uint8 | int8 | uint16 | int16 | uint32 | int32
      mask TypeOptions DataTypeDIDVar299: uint8 | int8 | uint16 | int16 | uint32 | int32
      mask TypeOptions DataTypeDIDVar300: uint8 | int8 | uint16 | int16 | uint32 | int32
      mask TypeOptions DataTypeDIDVar301: uint8 | int8 | uint16 | int16 | uint32 | int32
      mask TypeOptions DataTypeDIDVar302: uint8 | int8 | uint16 | int16 | uint32 | int32
      mask TypeOptions DataTypeDIDVar303: uint8 | int8 | uint16 | int16 | uint32 | int32
      mask TypeOptions DataTypeDIDVar304: uint8 | int8 | uint16 | int16 | uint32 | int32
      mask TypeOptions DataTypeDIDVar305: uint8 | int8 | uint16 | int16 | uint32 | int32
      mask TypeOptions DataTypeDIDVar306: uint8 | int8 | uint16 | int16 | uint32 | int32
      mask TypeOptions DataTypeDIDVar307: uint8 | int8 | uint16 | int16 | uint32 | int32
      mask TypeOptions DataTypeDIDVar308: uint8 | int8 | uint16 | int16 | uint32 | int32
      mask TypeOptions DataTypeDIDVar309: uint8 | int8 | uint16 | int16 | uint32 | int32
      mask TypeOptions DataTypeDIDVar310: uint8 | int8 | uint16 | int16 | uint32 | int32
      mask TypeOptions DataTypeDIDVar311: uint8 | int8 | uint16 | int16 | uint32 | int32
      mask TypeOptions DataTypeDIDVar312: uint8 | int8 | uint16 | int16 | uint32 | int32
      mask TypeOptions DataTypeDIDVar313: uint8 | int8 | uint16 | int16 | uint32 | int32
      mask TypeOptions DataTypeDIDVar314: uint8 | int8 | uint16 | int16 | uint32 | int32
      mask TypeOptions DataTypeDIDVar315: uint8 | int8 | uint16 | int16 | uint32 | int32
      mask TypeOptions DataTypeDIDVar316: uint8 | int8 | uint16 | int16 | uint32 | int32
      mask TypeOptions DataTypeDIDVar317: uint8 | int8 | uint16 | int16 | uint32 | int32
      mask TypeOptions DataTypeDIDVar318: uint8 | int8 | uint16 | int16 | uint32 | int32
      mask TypeOptions DataTypeDIDVar319: uint8 | int8 | uint16 | int16 | uint32 | int32
      mask TypeOptions DataTypeDIDVar320: uint8 | int8 | uint16 | int16 | uint32 | int32
      mask TypeOptions DataTypeDIDVar321: uint8 | int8 | uint16 | int16 | uint32 | int32
      mask TypeOptions DataTypeDIDVar322: uint8 | int8 | uint16 | int16 | uint32 | int32
      mask TypeOptions DataTypeDIDVar323: uint8 | int8 | uint16 | int16 | uint32 | int32
      mask TypeOptions DataTypeDIDVar324: uint8 | int8 | uint16 | int16 | uint32 | int32
      mask TypeOptions DataTypeDIDVar325: uint8 | int8 | uint16 | int16 | uint32 | int32
      mask TypeOptions DataTypeDIDVar326: uint8 | int8 | uint16 | int16 | uint32 | int32
      mask TypeOptions DataTypeDIDVar327: uint8 | int8 | uint16 | int16 | uint32 | int32
      mask TypeOptions DataTypeDIDVar328: uint8 | int8 | uint16 | int16 | uint32 | int32
      mask TypeOptions DataTypeDIDVar329: uint8 | int8 | uint16 | int16 | uint32 | int32
      mask TypeOptions DataTypeDIDVar330: uint8 | int8 | uint16 | int16 | uint32 | int32
      mask TypeOptions DataTypeDIDVar331: uint8 | int8 | uint16 | int16 | uint32 | int32
      mask TypeOptions DataTypeDIDVar332: uint8 | int8 | uint16 | int16 | uint32 | int32
      mask TypeOptions DataTypeDIDVar333: uint8 | int8 | uint16 | int16 | uint32 | int32
      mask TypeOptions DataTypeDIDVar334: uint8 | int8 | uint16 | int16 | uint32 | int32
      mask TypeOptions DataTypeDIDVar335: uint8 | int8 | uint16 | int16 | uint32 | int32
      mask TypeOptions DataTypeDIDVar336: uint8 | int8 | uint16 | int16 | uint32 | int32
      mask TypeOptions DataTypeDIDVar337: uint8 | int8 | uint16 | int16 | uint32 | int32
      mask TypeOptions DataTypeDIDVar338: uint8 | int8 | uint16 | int16 | uint32 | int32
      mask TypeOptions DataTypeDIDVar339: uint8 | int8 | uint16 | int16 | uint32 | int32
      mask TypeOptions DataTypeDIDVar340: uint8 | int8 | uint16 | int16 | uint32 | int32
      mask TypeOptions DataTypeDIDVar341: uint8 | int8 | uint16 | int16 | uint32 | int32
      mask TypeOptions DataTypeDIDVar342: uint8 | int8 | uint16 | int16 | uint32 | int32
      mask TypeOptions DataTypeDIDVar343: uint8 | int8 | uint16 | int16 | uint32 | int32
      mask TypeOptions DataTypeDIDVar344: uint8 | int8 | uint16 | int16 | uint32 | int32
      mask TypeOptions DataTypeDIDVar345: uint8 | int8 | uint16 | int16 | uint32 | int32
      mask TypeOptions DataTypeDIDVar346: uint8 | int8 | uint16 | int16 | uint32 | int32
      mask TypeOptions DataTypeDIDVar347: uint8 | int8 | uint16 | int16 | uint32 | int32
      mask TypeOptions DataTypeDIDVar348: uint8 | int8 | uint16 | int16 | uint32 | int32
      mask TypeOptions DataTypeDIDVar349: uint8 | int8 | uint16 | int16 | uint32 | int32
      mask TypeOptions DataTypeDIDVar350: uint8 | int8 | uint16 | int16 | uint32 | int32
      mask TypeOptions DataTypeDIDVar351: uint8 | int8 | uint16 | int16 | uint32 | int32
      mask TypeOptions DataTypeDIDVar352: uint8 | int8 | uint16 | int16 | uint32 | int32
      mask TypeOptions DataTypeDIDVar353: uint8 | int8 | uint16 | int16 | uint32 | int32
      mask TypeOptions DataTypeDIDVar354: uint8 | int8 | uint16 | int16 | uint32 | int32
      mask TypeOptions DataTypeDIDVar355: uint8 | int8 | uint16 | int16 | uint32 | int32
      mask TypeOptions DataTypeDIDVar356: uint8 | int8 | uint16 | int16 | uint32 | int32
      mask TypeOptions DataTypeDIDVar357: uint8 | int8 | uint16 | int16 | uint32 | int32
      mask TypeOptions DataTypeDIDVar358: uint8 | int8 | uint16 | int16 | uint32 | int32
      mask TypeOptions DataTypeDIDVar359: uint8 | int8 | uint16 | int16 | uint32 | int32
      mask TypeOptions DataTypeDIDVar360: uint8 | int8 | uint16 | int16 | uint32 | int32
      mask TypeOptions DataTypeDIDVar361: uint8 | int8 | uint16 | int16 | uint32 | int32
      mask TypeOptions DataTypeDIDVar362: uint8 | int8 | uint16 | int16 | uint32 | int32
      mask TypeOptions DataTypeDIDVar363: uint8 | int8 | uint16 | int16 | uint32 | int32
      mask TypeOptions DataTypeDIDVar364: uint8 | int8 | uint16 | int16 | uint32 | int32
      mask TypeOptions DataTypeDIDVar365: uint8 | int8 | uint16 | int16 | uint32 | int32
      mask TypeOptions DataTypeDIDVar366: uint8 | int8 | uint16 | int16 | uint32 | int32
      mask TypeOptions DataTypeDIDVar367: uint8 | int8 | uint16 | int16 | uint32 | int32
      mask TypeOptions DataTypeDIDVar368: uint8 | int8 | uint16 | int16 | uint32 | int32
      mask TypeOptions DataTypeDIDVar369: uint8 | int8 | uint16 | int16 | uint32 | int32
      mask TypeOptions DataTypeDIDVar370: uint8 | int8 | uint16 | int16 | uint32 | int32
      mask TypeOptions DataTypeDIDVar371: uint8 | int8 | uint16 | int16 | uint32 | int32
      mask TypeOptions DataTypeDIDVar372: uint8 | int8 | uint16 | int16 | uint32 | int32
      mask TypeOptions DataTypeDIDVar373: uint8 | int8 | uint16 | int16 | uint32 | int32
      mask TypeOptions DataTypeDIDVar374: uint8 | int8 | uint16 | int16 | uint32 | int32
      mask TypeOptions DataTypeDIDVar375: uint8 | int8 | uint16 | int16 | uint32 | int32
      mask TypeOptions DataTypeDIDVar376: uint8 | int8 | uint16 | int16 | uint32 | int32
      mask TypeOptions DataTypeDIDVar377: uint8 | int8 | uint16 | int16 | uint32 | int32
      mask TypeOptions DataTypeDIDVar378: uint8 | int8 | uint16 | int16 | uint32 | int32
      mask TypeOptions DataTypeDIDVar379: uint8 | int8 | uint16 | int16 | uint32 | int32
      mask TypeOptions DataTypeDIDVar380: uint8 | int8 | uint16 | int16 | uint32 | int32
      mask TypeOptions DataTypeDIDVar381: uint8 | int8 | uint16 | int16 | uint32 | int32
      mask TypeOptions DataTypeDIDVar382: uint8 | int8 | uint16 | int16 | uint32 | int32
      mask TypeOptions DataTypeDIDVar383: uint8 | int8 | uint16 | int16 | uint32 | int32
      mask TypeOptions DataTypeDIDVar384: uint8 | int8 | uint16 | int16 | uint32 | int32
      mask TypeOptions DataTypeDIDVar385: uint8 | int8 | uint16 | int16 | uint32 | int32
      mask TypeOptions DataTypeDIDVar386: uint8 | int8 | uint16 | int16 | uint32 | int32
      mask TypeOptions DataTypeDIDVar387: uint8 | int8 | uint16 | int16 | uint32 | int32
      mask TypeOptions DataTypeDIDVar388: uint8 | int8 | uint16 | int16 | uint32 | int32
      mask TypeOptions DataTypeDIDVar389: uint8 | int8 | uint16 | int16 | uint32 | int32
      mask TypeOptions DataTypeDIDVar390: uint8 | int8 | uint16 | int16 | uint32 | int32
      mask TypeOptions DataTypeDIDVar391: uint8 | int8 | uint16 | int16 | uint32 | int32
      mask TypeOptions DataTypeDIDVar392: uint8 | int8 | uint16 | int16 | uint32 | int32
      mask TypeOptions DataTypeDIDVar393: uint8 | int8 | uint16 | int16 | uint32 | int32
      mask TypeOptions DataTypeDIDVar394: uint8 | int8 | uint16 | int16 | uint32 | int32
      mask TypeOptions DataTypeDIDVar395: uint8 | int8 | uint16 | int16 | uint32 | int32
      mask TypeOptions DataTypeDIDVar396: uint8 | int8 | uint16 | int16 | uint32 | int32
      mask TypeOptions DataTypeDIDVar397: uint8 | int8 | uint16 | int16 | uint32 | int32
      mask TypeOptions DataTypeDIDVar398: uint8 | int8 | uint16 | int16 | uint32 | int32
      mask TypeOptions DataTypeDIDVar399: uint8 | int8 | uint16 | int16 | uint32 | int32
      mask TypeOptions DataTypeDIDVar400: uint8 | int8 | uint16 | int16 | uint32 | int32
  AEMS_DCM_DID_WRITEDATA : Subsystem  Tag=[LIB]  mask(AEMS_DCM_DID_WRITEDATA){ConfigManagement=1, DIDAbstract=DCM_DID_XXXX, NumDIDVar=1, DataType_DID_1=uint8, ResolDID_1=1, OffsetDID_1=0, OutVarName_1=DID_1, DataType_DID_2=int8, ResolDID_2=1, OffsetDID_2=0, OutVarName_2=DID_2, DataType_DID_3=int32, ResolDID_3=1, OffsetDID_3=0, OutVarName_3=DID_3, DataType_DID_4=uint16, ResolDID_4=1, OffsetDID_4=0, OutVarName_4=DID_4, DataType_DID_5=int8, ResolDID_5=1, OffsetDID_5=0, OutVarName_5=DID_5, DataType_DID_6=int8, ResolDID_6=1, OffsetDID_6=0, OutVarName_6=DID_6, DataType_DID_7=int8, ResolDID_7=1, OffsetDID_7=0, OutVarName_7=DID_7, DataType_DID_8=int8, ResolDID_8=1, OffsetDID_8=0, OutVarName_8=DID_8, DataType_DID_9=int8, ResolDID_9=1, OffsetDID_9=0, OutVarName_9=DID_9, DataType_DID_10=int8, ResolDID_10=1, OffsetDID_10=0, OutVarName_10=DID_10, DataType_DID_11=int8, ResolDID_11=1, OffsetDID_11=0, OutVarName_11=DID_11, DataType_DID_12=int8, ResolDID_12=1, OffsetDID_12=0, OutVarName_12=DID_12, DataType_DID_13=int8, ResolDID_13=1, OffsetDID_13=0, OutVarName_13=DID_13, DataType_DID_14=int8, ResolDID_14=1, OffsetDID_14=0, OutVarName_14=DID_14, DataType_DID_15=int8, ResolDID_15=1, OffsetDID_15=0, OutVarName_15=DID_15, DataType_DID_16=int8, ResolDID_16=1, OffsetDID_16=0, OutVarName_16=DID_16, DataType_DID_17=int8, ResolDID_17=1, OffsetDID_17=0, OutVarName_17=DID_17, DataType_DID_18=int8, ResolDID_18=1, OffsetDID_18=0, OutVarName_18=DID_18, DataType_DID_19=int8, ResolDID_19=1, OffsetDID_19=0, OutVarName_19=DID_19, DataType_DID_20=int8, ResolDID_20=1, OffsetDID_20=0, OutVarName_20=DID_20, DataType_DID_21=int8, ResolDID_21=1, OffsetDID_21=0, OutVarName_21=DID_21, DataType_DID_22=int8, ResolDID_22=1, OffsetDID_22=0, OutVarName_22=DID_22, DataType_DID_23=int8, ResolDID_23=1, OffsetDID_23=0, OutVarName_23=DID_23, DataType_DID_24=int8, ResolDID_24=1, OffsetDID_24=0, OutVarName_24=DID_24, DataType_DID_25=int8, ResolDID_25=1, OffsetDID_25=0, OutVarName_25=DID_25, DataType_DID_26=int8, ResolDID_26=1, OffsetDID_26=0, OutVarName_26=DID_26, DataType_DID_27=int8, ResolDID_27=1, OffsetDID_27=0, OutVarName_27=DID_27, DataType_DID_28=int8, ResolDID_28=1, OffsetDID_28=0, OutVarName_28=DID_28, DataType_DID_29=int8, ResolDID_29=1, OffsetDID_29=0, OutVarName_29=DID_29, DataType_DID_30=int8, ResolDID_30=1, OffsetDID_30=0, OutVarName_30=DID_30, DataType_DID_31=int8, ResolDID_31=1, OffsetDID_31=0, OutVarName_31=DID_31, DataType_DID_32=int8, ResolDID_32=1, OffsetDID_32=0, OutVarName_32=DID_32, DataType_DID_33=int8, ResolDID_33=1, OffsetDID_33=0, OutVarName_33=DID_33, DataType_DID_34=int8, ResolDID_34=1, OffsetDID_34=0, OutVarName_34=DID_34, DataType_DID_35=int8, ResolDID_35=1, OffsetDID_35=0, OutVarName_35=DID_35, DataType_DID_36=int8, ResolDID_36=1, OffsetDID_36=0, OutVarName_36=DID_36, DataType_DID_37=int8, ResolDID_37=1, OffsetDID_37=0, OutVarName_37=DID_37, DataType_DID_38=int8, ResolDID_38=1, OffsetDID_38=0, OutVarName_38=DID_38, DataType_DID_39=int8, ResolDID_39=1, OffsetDID_39=0, OutVarName_39=DID_39, DataType_DID_40=int8, ResolDID_40=1, OffsetDID_40=0, OutVarName_40=DID_40, DataType_DID_41=int8, ResolDID_41=1, OffsetDID_41=0, OutVarName_41=DID_41, DataType_DID_42=int8, ResolDID_42=1, OffsetDID_42=0, OutVarName_42=DID_42, DataType_DID_43=int8, ResolDID_43=1, OffsetDID_43=0, OutVarName_43=DID_43, DataType_DID_44=int8, ResolDID_44=1, OffsetDID_44=0, OutVarName_44=DID_44, DataType_DID_45=int8, ResolDID_45=1, OffsetDID_45=0, OutVarName_45=DID_45, DataType_DID_46=int8, ResolDID_46=1, OffsetDID_46=0, OutVarName_46=DID_46, DataType_DID_47=int8, ResolDID_47=1, OffsetDID_47=0, OutVarName_47=DID_47, DataType_DID_48=int8, ResolDID_48=1, OffsetDID_48=0, OutVarName_48=DID_48, DataType_DID_49=int8, ResolDID_49=1, OffsetDID_49=0, OutVarName_49=DID_49, DataType_DID_50=int8, ResolDID_50=1, OffsetDID_50=0, OutVarName_50=DID_50, DataType_DID_51=int8, ResolDID_51=1, OffsetDID_51=0, OutVarName_51=DID_51, DataType_DID_52=int8, ResolDID_52=1, OffsetDID_52=0, OutVarName_52=DID_52, DataType_DID_53=int8, ResolDID_53=1, OffsetDID_53=0, OutVarName_53=DID_53, DataType_DID_54=int8, ResolDID_54=1, OffsetDID_54=0, OutVarName_54=DID_54, DataType_DID_55=int8, ResolDID_55=1, OffsetDID_55=0, OutVarName_55=DID_55, DataType_DID_56=int8, ResolDID_56=1, OffsetDID_56=0, OutVarName_56=DID_56, DataType_DID_57=int8, ResolDID_57=1, OffsetDID_57=0, OutVarName_57=DID_57, DataType_DID_58=int8, ResolDID_58=1, OffsetDID_58=0, OutVarName_58=DID_58, DataType_DID_59=int8, ResolDID_59=1, OffsetDID_59=0, OutVarName_59=DID_59, DataType_DID_60=int8, ResolDID_60=1, OffsetDID_60=0, OutVarName_60=DID_60, DataType_DID_61=int8, ResolDID_61=1, OffsetDID_61=0, OutVarName_61=DID_61, DataType_DID_62=int8, ResolDID_62=1, OffsetDID_62=0, OutVarName_62=DID_62, DataType_DID_63=int8, ResolDID_63=1, OffsetDID_63=0, OutVarName_63=DID_63, DataType_DID_64=int8, ResolDID_64=1, OffsetDID_64=0, OutVarName_64=DID_64, DataType_DID_65=int8, ResolDID_65=1, OffsetDID_65=0, OutVarName_65=DID_65, DataType_DID_66=int8, ResolDID_66=1, OffsetDID_66=0, OutVarName_66=DID_66, DataType_DID_67=int8, ResolDID_67=1, OffsetDID_67=0, OutVarName_67=DID_67, DataType_DID_68=int8, ResolDID_68=1, OffsetDID_68=0, OutVarName_68=DID_68, DataType_DID_69=int8, ResolDID_69=1, OffsetDID_69=0, OutVarName_69=DID_69, DataType_DID_70=int8, ResolDID_70=1, OffsetDID_70=0, OutVarName_70=DID_70, DataType_DID_71=int8, ResolDID_71=1, OffsetDID_71=0, OutVarName_71=DID_71, DataType_DID_72=int8, ResolDID_72=1, OffsetDID_72=0, OutVarName_72=DID_72, DataType_DID_73=int8, ResolDID_73=1, OffsetDID_73=0, OutVarName_73=DID_73, DataType_DID_74=int8, ResolDID_74=1, OffsetDID_74=0, OutVarName_74=DID_74, DataType_DID_75=int8, ResolDID_75=1, OffsetDID_75=0, OutVarName_75=DID_75, DataType_DID_76=int8, ResolDID_76=1, OffsetDID_76=0, OutVarName_76=DID_76, DataType_DID_77=int8, ResolDID_77=1, OffsetDID_77=0, OutVarName_77=DID_77, DataType_DID_78=int8, ResolDID_78=1, OffsetDID_78=0, OutVarName_78=DID_78, DataType_DID_79=int8, ResolDID_79=1, OffsetDID_79=0, OutVarName_79=DID_79, DataType_DID_80=int8, ResolDID_80=1, OffsetDID_80=0, OutVarName_80=DID_80, DataType_DID_81=int8, ResolDID_81=1, OffsetDID_81=0, OutVarName_81=DID_81, DataType_DID_82=int8, ResolDID_82=1, OffsetDID_82=0, OutVarName_82=DID_82, DataType_DID_83=int8, ResolDID_83=1, OffsetDID_83=0, OutVarName_83=DID_83, DataType_DID_84=int8, ResolDID_84=1, OffsetDID_84=0, OutVarName_84=DID_84, DataType_DID_85=int8, ResolDID_85=1, OffsetDID_85=0, OutVarName_85=DID_85, DataType_DID_86=int8, ResolDID_86=1, OffsetDID_86=0, OutVarName_86=DID_86, DataType_DID_87=int8, ResolDID_87=1, OffsetDID_87=0, OutVarName_87=DID_87, DataType_DID_88=int8, ResolDID_88=1, OffsetDID_88=0, OutVarName_88=DID_88, DataType_DID_89=int8, ResolDID_89=1, OffsetDID_89=0, OutVarName_89=DID_89, DataType_DID_90=int8, ResolDID_90=1, OffsetDID_90=0, OutVarName_90=DID_90, DataType_DID_91=int8, ResolDID_91=1, OffsetDID_91=0, OutVarName_91=DID_91, DataType_DID_92=int8, ResolDID_92=1, OffsetDID_92=0, OutVarName_92=DID_92, DataType_DID_93=int8, ResolDID_93=1, OffsetDID_93=0, OutVarName_93=DID_93, DataType_DID_94=int8, ResolDID_94=1, OffsetDID_94=0, OutVarName_94=DID_94, DataType_DID_95=int8, ResolDID_95=1, OffsetDID_95=0, OutVarName_95=DID_95, DataType_DID_96=int8, ResolDID_96=1, OffsetDID_96=0, OutVarName_96=DID_96, DataType_DID_97=int8, ResolDID_97=1, OffsetDID_97=0, OutVarName_97=DID_97, DataType_DID_98=int8, ResolDID_98=1, OffsetDID_98=0, OutVarName_98=DID_98, DataType_DID_99=int8, ResolDID_99=1, OffsetDID_99=0, OutVarName_99=DID_99, DataType_DID_100=int8, ResolDID_100=1, OffsetDID_100=0, OutVarName_100=DID_100, DataType_DID_101=int8, ResolDID_101=1, OffsetDID_101=0, OutVarName_101=DID_101, DataType_DID_102=int8, ResolDID_102=1, OffsetDID_102=0, OutVarName_102=DID_102, DataType_DID_103=int8, ResolDID_103=1, OffsetDID_103=0, OutVarName_103=DID_103, DataType_DID_104=int8, ResolDID_104=1, OffsetDID_104=0, OutVarName_104=DID_104, DataType_DID_105=int8, ResolDID_105=1, OffsetDID_105=0, OutVarName_105=DID_105, DataType_DID_106=int8, ResolDID_106=1, OffsetDID_106=0, OutVarName_106=DID_106, DataType_DID_107=int8, ResolDID_107=1, OffsetDID_107=0, OutVarName_107=DID_107, DataType_DID_108=int8, ResolDID_108=1, OffsetDID_108=0, OutVarName_108=DID_108, DataType_DID_109=int8, ResolDID_109=1, OffsetDID_109=0, OutVarName_109=DID_109, DataType_DID_110=int8, ResolDID_110=1, OffsetDID_110=0, OutVarName_110=DID_110, DataType_DID_111=int8, ResolDID_111=1, OffsetDID_111=0, OutVarName_111=DID_111, DataType_DID_112=int8, ResolDID_112=1, OffsetDID_112=0, OutVarName_112=DID_112, DataType_DID_113=int8, ResolDID_113=1, OffsetDID_113=0, OutVarName_113=DID_113, DataType_DID_114=int8, ResolDID_114=1, OffsetDID_114=0, OutVarName_114=DID_114, DataType_DID_115=int8, ResolDID_115=1, OffsetDID_115=0, OutVarName_115=DID_115, DataType_DID_116=int8, ResolDID_116=1, OffsetDID_116=0, OutVarName_116=DID_116, DataType_DID_117=int8, ResolDID_117=1, OffsetDID_117=0, OutVarName_117=DID_117, DataType_DID_118=int8, ResolDID_118=1, OffsetDID_118=0, OutVarName_118=DID_118, DataType_DID_119=int8, ResolDID_119=1, OffsetDID_119=0, OutVarName_119=DID_119, DataType_DID_120=int8, ResolDID_120=1, OffsetDID_120=0, OutVarName_120=DID_120, DataType_DID_121=int8, ResolDID_121=1, OffsetDID_121=0, OutVarName_121=DID_121, DataType_DID_122=int8, ResolDID_122=1, OffsetDID_122=0, OutVarName_122=DID_122, DataType_DID_123=int8, ResolDID_123=1, OffsetDID_123=0, OutVarName_123=DID_123, DataType_DID_124=int8, ResolDID_124=1, OffsetDID_124=0, OutVarName_124=DID_124, DataType_DID_125=int8, ResolDID_125=1, OffsetDID_125=0, OutVarName_125=DID_125, DataType_DID_126=int8, ResolDID_126=1, OffsetDID_126=0, OutVarName_126=DID_126, DataType_DID_127=int8, ResolDID_127=1, OffsetDID_127=0, OutVarName_127=DID_127, DataType_DID_128=int8, ResolDID_128=1, OffsetDID_128=0, OutVarName_128=DID_128, DataType_DID_129=int8, ResolDID_129=1, OffsetDID_129=0, OutVarName_129=DID_129, DataType_DID_130=int8, ResolDID_130=1, OffsetDID_130=0, OutVarName_130=DID_130, DataType_DID_131=int8, ResolDID_131=1, OffsetDID_131=0, OutVarName_131=DID_131, DataType_DID_132=int8, ResolDID_132=1, OffsetDID_132=0, OutVarName_132=DID_132, DataType_DID_133=int8, ResolDID_133=1, OffsetDID_133=0, OutVarName_133=DID_133, DataType_DID_134=int8, ResolDID_134=1, OffsetDID_134=0, OutVarName_134=DID_134, DataType_DID_135=int8, ResolDID_135=1, OffsetDID_135=0, OutVarName_135=DID_135, DataType_DID_136=int8, ResolDID_136=1, OffsetDID_136=0, OutVarName_136=DID_136, DataType_DID_137=int8, ResolDID_137=1, OffsetDID_137=0, OutVarName_137=DID_137, DataType_DID_138=int8, ResolDID_138=1, OffsetDID_138=0, OutVarName_138=DID_138, DataType_DID_139=int8, ResolDID_139=1, OffsetDID_139=0, OutVarName_139=DID_139, DataType_DID_140=int8, ResolDID_140=1, OffsetDID_140=0, OutVarName_140=DID_140, DataType_DID_141=int8, ResolDID_141=1, OffsetDID_141=0, OutVarName_141=DID_141, DataType_DID_142=int8, ResolDID_142=1, OffsetDID_142=0, OutVarName_142=DID_142, DataType_DID_143=int8, ResolDID_143=1, OffsetDID_143=0, OutVarName_143=DID_143, DataType_DID_144=int8, ResolDID_144=1, OffsetDID_144=0, OutVarName_144=DID_144, DataType_DID_145=int8, ResolDID_145=1, OffsetDID_145=0, OutVarName_145=DID_145, DataType_DID_146=int8, ResolDID_146=1, OffsetDID_146=0, OutVarName_146=DID_146, DataType_DID_147=int8, ResolDID_147=1, OffsetDID_147=0, OutVarName_147=DID_147, DataType_DID_148=int8, ResolDID_148=1, OffsetDID_148=0, OutVarName_148=DID_148, DataType_DID_149=int8, ResolDID_149=1, OffsetDID_149=0, OutVarName_149=DID_149, DataType_DID_150=int8, ResolDID_150=1, OffsetDID_150=0, OutVarName_150=DID_150, DataType_DID_151=int8, ResolDID_151=1, OffsetDID_151=0, OutVarName_151=DID_151, DataType_DID_152=int8, ResolDID_152=1, OffsetDID_152=0, OutVarName_152=DID_152, DataType_DID_153=int8, ResolDID_153=1, OffsetDID_153=0, OutVarName_153=DID_153, DataType_DID_154=int8, ResolDID_154=1, OffsetDID_154=0, OutVarName_154=DID_154, DataType_DID_155=int8, ResolDID_155=1, OffsetDID_155=0, OutVarName_155=DID_155, DataType_DID_156=int8, ResolDID_156=1, OffsetDID_156=0, OutVarName_156=DID_156, DataType_DID_157=int8, ResolDID_157=1, OffsetDID_157=0, OutVarName_157=DID_157, DataType_DID_158=int8, ResolDID_158=1, OffsetDID_158=0, OutVarName_158=DID_158, DataType_DID_159=int8, ResolDID_159=1, OffsetDID_159=0, OutVarName_159=DID_159, DataType_DID_160=int8, ResolDID_160=1, OffsetDID_160=0, OutVarName_160=DID_160, DataType_DID_161=int8, ResolDID_161=1, OffsetDID_161=0, OutVarName_161=DID_161, DataType_DID_162=int8, ResolDID_162=1, OffsetDID_162=0, OutVarName_162=DID_162, DataType_DID_163=int8, ResolDID_163=1, OffsetDID_163=0, OutVarName_163=DID_163, DataType_DID_164=int8, ResolDID_164=1, OffsetDID_164=0, OutVarName_164=DID_164, DataType_DID_165=int8, ResolDID_165=1, OffsetDID_165=0, OutVarName_165=DID_165, DataType_DID_166=int8, ResolDID_166=1, OffsetDID_166=0, OutVarName_166=DID_166, DataType_DID_167=int8, ResolDID_167=1, OffsetDID_167=0, OutVarName_167=DID_167, DataType_DID_168=int8, ResolDID_168=1, OffsetDID_168=0, OutVarName_168=DID_168, DataType_DID_169=int8, ResolDID_169=1, OffsetDID_169=0, OutVarName_169=DID_169, DataType_DID_170=int8, ResolDID_170=1, OffsetDID_170=0, OutVarName_170=DID_170, DataType_DID_171=int8, ResolDID_171=1, OffsetDID_171=0, OutVarName_171=DID_171, DataType_DID_172=int8, ResolDID_172=1, OffsetDID_172=0, OutVarName_172=DID_172, DataType_DID_173=int8, ResolDID_173=1, OffsetDID_173=0, OutVarName_173=DID_173, DataType_DID_174=int8, ResolDID_174=1, OffsetDID_174=0, OutVarName_174=DID_174, DataType_DID_175=int8, ResolDID_175=1, OffsetDID_175=0, OutVarName_175=DID_175, DataType_DID_176=int8, ResolDID_176=1, OffsetDID_176=0, OutVarName_176=DID_176, DataType_DID_177=int8, ResolDID_177=1, OffsetDID_177=0, OutVarName_177=DID_177, DataType_DID_178=int8, ResolDID_178=1, OffsetDID_178=0, OutVarName_178=DID_178, DataType_DID_179=int8, ResolDID_179=1, OffsetDID_179=0, OutVarName_179=DID_179, DataType_DID_180=int8, ResolDID_180=1, OffsetDID_180=0, OutVarName_180=DID_180, DataType_DID_181=int8, ResolDID_181=1, OffsetDID_181=0, OutVarName_181=DID_181, DataType_DID_182=int8, ResolDID_182=1, OffsetDID_182=0, OutVarName_182=DID_182, DataType_DID_183=int8, ResolDID_183=1, OffsetDID_183=0, OutVarName_183=DID_183, DataType_DID_184=int8, ResolDID_184=1, OffsetDID_184=0, OutVarName_184=DID_184, DataType_DID_185=int8, ResolDID_185=1, OffsetDID_185=0, OutVarName_185=DID_185, DataType_DID_186=int8, ResolDID_186=1, OffsetDID_186=0, OutVarName_186=DID_186, DataType_DID_187=int8, ResolDID_187=1, OffsetDID_187=0, OutVarName_187=DID_187, DataType_DID_188=int8, ResolDID_188=1, OffsetDID_188=0, OutVarName_188=DID_188, DataType_DID_189=int8, ResolDID_189=1, OffsetDID_189=0, OutVarName_189=DID_189, DataType_DID_190=int8, ResolDID_190=1, OffsetDID_190=0, OutVarName_190=DID_190, DataType_DID_191=int8, ResolDID_191=1, OffsetDID_191=0, OutVarName_191=DID_191, DataType_DID_192=int8, ResolDID_192=1, OffsetDID_192=0, OutVarName_192=DID_192, DataType_DID_193=int8, ResolDID_193=1, OffsetDID_193=0, OutVarName_193=DID_193, DataType_DID_194=int8, ResolDID_194=1, OffsetDID_194=0, OutVarName_194=DID_194, DataType_DID_195=int8, ResolDID_195=1, OffsetDID_195=0, OutVarName_195=DID_195, DataType_DID_196=int8, ResolDID_196=1, OffsetDID_196=0, OutVarName_196=DID_196, DataType_DID_197=int8, ResolDID_197=1, OffsetDID_197=0, OutVarName_197=DID_197, DataType_DID_198=int8, ResolDID_198=1, OffsetDID_198=0, OutVarName_198=DID_198, DataType_DID_199=int8, ResolDID_199=1, OffsetDID_199=0, OutVarName_199=DID_199, DataType_DID_200=int8, ResolDID_200=1, OffsetDID_200=0, OutVarName_200=DID_200, DataType_DID_201=int8, ResolDID_201=1, OffsetDID_201=0, OutVarName_201=DID_201, DataType_DID_202=int8, ResolDID_202=1, OffsetDID_202=0, OutVarName_202=DID_202, DataType_DID_203=int8, ResolDID_203=1, OffsetDID_203=0, OutVarName_203=DID_203, DataType_DID_204=int8, ResolDID_204=1, OffsetDID_204=0, OutVarName_204=DID_204, DataType_DID_205=int8, ResolDID_205=1, OffsetDID_205=0, OutVarName_205=DID_205, DataType_DID_206=int8, ResolDID_206=1, OffsetDID_206=0, OutVarName_206=DID_206, DataType_DID_207=int8, ResolDID_207=1, OffsetDID_207=0, OutVarName_207=DID_207, DataType_DID_208=int8, ResolDID_208=1, OffsetDID_208=0, OutVarName_208=DID_208, DataType_DID_209=int8, ResolDID_209=1, OffsetDID_209=0, OutVarName_209=DID_209, DataType_DID_210=int8, ResolDID_210=1, OffsetDID_210=0, OutVarName_210=DID_210, DataType_DID_211=int8, ResolDID_211=1, OffsetDID_211=0, OutVarName_211=DID_211, DataType_DID_212=int8, ResolDID_212=1, OffsetDID_212=0, OutVarName_212=DID_212, DataType_DID_213=int8, ResolDID_213=1, OffsetDID_213=0, OutVarName_213=DID_213, DataType_DID_214=int8, ResolDID_214=1, OffsetDID_214=0, OutVarName_214=DID_214, DataType_DID_215=int8, ResolDID_215=1, OffsetDID_215=0, OutVarName_215=DID_215, DataType_DID_216=int8, ResolDID_216=1, OffsetDID_216=0, OutVarName_216=DID_216, DataType_DID_217=int8, ResolDID_217=1, OffsetDID_217=0, OutVarName_217=DID_217, DataType_DID_218=int8, ResolDID_218=1, OffsetDID_218=0, OutVarName_218=DID_218, DataType_DID_219=int8, ResolDID_219=1, OffsetDID_219=0, OutVarName_219=DID_219, DataType_DID_220=int8, ResolDID_220=1, OffsetDID_220=0, OutVarName_220=DID_220, DataType_DID_221=int8, ResolDID_221=1, OffsetDID_221=0, OutVarName_221=DID_221, DataType_DID_222=int8, ResolDID_222=1, OffsetDID_222=0, OutVarName_222=DID_222, DataType_DID_223=int8, ResolDID_223=1, OffsetDID_223=0, OutVarName_223=DID_223, DataType_DID_224=int8, ResolDID_224=1, OffsetDID_224=0, OutVarName_224=DID_224, DataType_DID_225=int8, ResolDID_225=1, OffsetDID_225=0, OutVarName_225=DID_225, DataType_DID_226=int8, ResolDID_226=1, OffsetDID_226=0, OutVarName_226=DID_226, DataType_DID_227=int8, ResolDID_227=1, OffsetDID_227=0, OutVarName_227=DID_227, DataType_DID_228=int8, ResolDID_228=1, OffsetDID_228=0, OutVarName_228=DID_228, DataType_DID_229=int8, ResolDID_229=1, OffsetDID_229=0, OutVarName_229=DID_229, DataType_DID_230=int8, ResolDID_230=1, OffsetDID_230=0, OutVarName_230=DID_230, DataType_DID_231=int8, ResolDID_231=1, OffsetDID_231=0, OutVarName_231=DID_231, DataType_DID_232=int8, ResolDID_232=1, OffsetDID_232=0, OutVarName_232=DID_232, DataType_DID_233=int8, ResolDID_233=1, OffsetDID_233=0, OutVarName_233=DID_233, DataType_DID_234=int8, ResolDID_234=1, OffsetDID_234=0, OutVarName_234=DID_234, DataType_DID_235=int8, ResolDID_235=1, OffsetDID_235=0, OutVarName_235=DID_235, DataType_DID_236=int8, ResolDID_236=1, OffsetDID_236=0, OutVarName_236=DID_236, DataType_DID_237=int8, ResolDID_237=1, OffsetDID_237=0, OutVarName_237=DID_237, DataType_DID_238=int8, ResolDID_238=1, OffsetDID_238=0, OutVarName_238=DID_238, DataType_DID_239=int8, ResolDID_239=1, OffsetDID_239=0, OutVarName_239=DID_239, DataType_DID_240=int8, ResolDID_240=1, OffsetDID_240=0, OutVarName_240=DID_240, DataType_DID_241=int8, ResolDID_241=1, OffsetDID_241=0, OutVarName_241=DID_241, DataType_DID_242=int8, ResolDID_242=1, OffsetDID_242=0, OutVarName_242=DID_242, DataType_DID_243=int8, ResolDID_243=1, OffsetDID_243=0, OutVarName_243=DID_243, DataType_DID_244=int8, ResolDID_244=1, OffsetDID_244=0, OutVarName_244=DID_244, DataType_DID_245=int8, ResolDID_245=1, OffsetDID_245=0, OutVarName_245=DID_245, DataType_DID_246=int8, ResolDID_246=1, OffsetDID_246=0, OutVarName_246=DID_246, DataType_DID_247=int8, ResolDID_247=1, OffsetDID_247=0, OutVarName_247=DID_247, DataType_DID_248=int8, ResolDID_248=1, OffsetDID_248=0, OutVarName_248=DID_248, DataType_DID_249=int8, ResolDID_249=1, OffsetDID_249=0, OutVarName_249=DID_249, DataType_DID_250=int8, ResolDID_250=1, OffsetDID_250=0, OutVarName_250=DID_250, DataType_DID_251=int8, ResolDID_251=1, OffsetDID_251=0, OutVarName_251=DID_251, DataType_DID_252=int8, ResolDID_252=1, OffsetDID_252=0, OutVarName_252=DID_252, DataType_DID_253=int8, ResolDID_253=1, OffsetDID_253=0, OutVarName_253=DID_253, DataType_DID_254=int8, ResolDID_254=1, OffsetDID_254=0, OutVarName_254=DID_254, DataType_DID_255=int8, ResolDID_255=1, OffsetDID_255=0, OutVarName_255=DID_255, DataType_DID_256=int8, ResolDID_256=1, OffsetDID_256=0, OutVarName_256=DID_256, DataType_DID_257=int8, ResolDID_257=1, OffsetDID_257=0, OutVarName_257=DID_257, DataType_DID_258=int8, ResolDID_258=1, OffsetDID_258=0, OutVarName_258=DID_258, DataType_DID_259=int8, ResolDID_259=1, OffsetDID_259=0, OutVarName_259=DID_259, DataType_DID_260=int8, ResolDID_260=1, OffsetDID_260=0, OutVarName_260=DID_260, DataType_DID_261=int8, ResolDID_261=1, OffsetDID_261=0, OutVarName_261=DID_261, DataType_DID_262=int8, ResolDID_262=1, OffsetDID_262=0, OutVarName_262=DID_262, DataType_DID_263=int8, ResolDID_263=1, OffsetDID_263=0, OutVarName_263=DID_263, DataType_DID_264=int8, ResolDID_264=1, OffsetDID_264=0, OutVarName_264=DID_264, DataType_DID_265=int8, ResolDID_265=1, OffsetDID_265=0, OutVarName_265=DID_265, DataType_DID_266=int8, ResolDID_266=1, OffsetDID_266=0, OutVarName_266=DID_266, DataType_DID_267=int8, ResolDID_267=1, OffsetDID_267=0, OutVarName_267=DID_267, DataType_DID_268=int8, ResolDID_268=1, OffsetDID_268=0, OutVarName_268=DID_268, DataType_DID_269=int8, ResolDID_269=1, OffsetDID_269=0, OutVarName_269=DID_269, DataType_DID_270=int8, ResolDID_270=1, OffsetDID_270=0, OutVarName_270=DID_270, DataType_DID_271=int8, ResolDID_271=1, OffsetDID_271=0, OutVarName_271=DID_271, DataType_DID_272=int8, ResolDID_272=1, OffsetDID_272=0, OutVarName_272=DID_272, DataType_DID_273=int8, ResolDID_273=1, OffsetDID_273=0, OutVarName_273=DID_273, DataType_DID_274=int8, ResolDID_274=1, OffsetDID_274=0, OutVarName_274=DID_274, DataType_DID_275=int8, ResolDID_275=1, OffsetDID_275=0, OutVarName_275=DID_275, DataType_DID_276=int8, ResolDID_276=1, OffsetDID_276=0, OutVarName_276=DID_276, DataType_DID_277=int8, ResolDID_277=1, OffsetDID_277=0, OutVarName_277=DID_277, DataType_DID_278=int8, ResolDID_278=1, OffsetDID_278=0, OutVarName_278=DID_278, DataType_DID_279=int8, ResolDID_279=1, OffsetDID_279=0, OutVarName_279=DID_279, DataType_DID_280=int8, ResolDID_280=1, OffsetDID_280=0, OutVarName_280=DID_280, DataType_DID_281=int8, ResolDID_281=1, OffsetDID_281=0, OutVarName_281=DID_281, DataType_DID_282=int8, ResolDID_282=1, OffsetDID_282=0, OutVarName_282=DID_282, DataType_DID_283=int8, ResolDID_283=1, OffsetDID_283=0, OutVarName_283=DID_283, DataType_DID_284=int8, ResolDID_284=1, OffsetDID_284=0, OutVarName_284=DID_284, DataType_DID_285=int8, ResolDID_285=1, OffsetDID_285=0, OutVarName_285=DID_285, DataType_DID_286=int8, ResolDID_286=1, OffsetDID_286=0, OutVarName_286=DID_286, DataType_DID_287=int8, ResolDID_287=1, OffsetDID_287=0, OutVarName_287=DID_287, DataType_DID_288=int8, ResolDID_288=1, OffsetDID_288=0, OutVarName_288=DID_288, DataType_DID_289=int8, ResolDID_289=1, OffsetDID_289=0, OutVarName_289=DID_289, DataType_DID_290=int8, ResolDID_290=1, OffsetDID_290=0, OutVarName_290=DID_290, DataType_DID_291=int8, ResolDID_291=1, OffsetDID_291=0, OutVarName_291=DID_291, DataType_DID_292=int8, ResolDID_292=1, OffsetDID_292=0, OutVarName_292=DID_292, DataType_DID_293=int8, ResolDID_293=1, OffsetDID_293=0, OutVarName_293=DID_293, DataType_DID_294=int8, ResolDID_294=1, OffsetDID_294=0, OutVarName_294=DID_294, DataType_DID_295=int8, ResolDID_295=1, OffsetDID_295=0, OutVarName_295=DID_295, DataType_DID_296=int8, ResolDID_296=1, OffsetDID_296=0, OutVarName_296=DID_296, DataType_DID_297=int8, ResolDID_297=1, OffsetDID_297=0, OutVarName_297=DID_297, DataType_DID_298=int8, ResolDID_298=1, OffsetDID_298=0, OutVarName_298=DID_298, DataType_DID_299=int8, ResolDID_299=1, OffsetDID_299=0, OutVarName_299=DID_299, DataType_DID_300=int8, ResolDID_300=1, OffsetDID_300=0, OutVarName_300=DID_300, DataType_DID_301=int8, ResolDID_301=1, OffsetDID_301=0, OutVarName_301=DID_301, DataType_DID_302=int8, ResolDID_302=1, OffsetDID_302=0, OutVarName_302=DID_302, DataType_DID_303=int8, ResolDID_303=1, OffsetDID_303=0, OutVarName_303=DID_303, DataType_DID_304=int8, ResolDID_304=1, OffsetDID_304=0, OutVarName_304=DID_304, DataType_DID_305=int8, ResolDID_305=1, OffsetDID_305=0, OutVarName_305=DID_305, DataType_DID_306=int8, ResolDID_306=1, OffsetDID_306=0, OutVarName_306=DID_306, DataType_DID_307=int8, ResolDID_307=1, OffsetDID_307=0, OutVarName_307=DID_307, DataType_DID_308=int8, ResolDID_308=1, OffsetDID_308=0, OutVarName_308=DID_308, DataType_DID_309=int8, ResolDID_309=1, OffsetDID_309=0, OutVarName_309=DID_309, DataType_DID_310=int8, ResolDID_310=1, OffsetDID_310=0, OutVarName_310=DID_310, DataType_DID_311=int8, ResolDID_311=1, OffsetDID_311=0, OutVarName_311=DID_311, DataType_DID_312=int8, ResolDID_312=1, OffsetDID_312=0, OutVarName_312=DID_312, DataType_DID_313=int8, ResolDID_313=1, OffsetDID_313=0, OutVarName_313=DID_313, DataType_DID_314=int8, ResolDID_314=1, OffsetDID_314=0, OutVarName_314=DID_314, DataType_DID_315=int8, ResolDID_315=1, OffsetDID_315=0, OutVarName_315=DID_315, DataType_DID_316=int8, ResolDID_316=1, OffsetDID_316=0, OutVarName_316=DID_316, DataType_DID_317=int8, ResolDID_317=1, OffsetDID_317=0, OutVarName_317=DID_317, DataType_DID_318=int8, ResolDID_318=1, OffsetDID_318=0, OutVarName_318=DID_318, DataType_DID_319=int8, ResolDID_319=1, OffsetDID_319=0, OutVarName_319=DID_319, DataType_DID_320=int8, ResolDID_320=1, OffsetDID_320=0, OutVarName_320=DID_320, DataType_DID_321=int8, ResolDID_321=1, OffsetDID_321=0, OutVarName_321=DID_321, DataType_DID_322=int8, ResolDID_322=1, OffsetDID_322=0, OutVarName_322=DID_322, DataType_DID_323=int8, ResolDID_323=1, OffsetDID_323=0, OutVarName_323=DID_323, DataType_DID_324=int8, ResolDID_324=1, OffsetDID_324=0, OutVarName_324=DID_324, DataType_DID_325=int8, ResolDID_325=1, OffsetDID_325=0, OutVarName_325=DID_325, DataType_DID_326=int8, ResolDID_326=1, OffsetDID_326=0, OutVarName_326=DID_326, DataType_DID_327=int8, ResolDID_327=1, OffsetDID_327=0, OutVarName_327=DID_327, DataType_DID_328=int8, ResolDID_328=1, OffsetDID_328=0, OutVarName_328=DID_328, DataType_DID_329=int8, ResolDID_329=1, OffsetDID_329=0, OutVarName_329=DID_329, DataType_DID_330=int8, ResolDID_330=1, OffsetDID_330=0, OutVarName_330=DID_330, DataType_DID_331=int8, ResolDID_331=1, OffsetDID_331=0, OutVarName_331=DID_331, DataType_DID_332=int8, ResolDID_332=1, OffsetDID_332=0, OutVarName_332=DID_332, DataType_DID_333=int8, ResolDID_333=1, OffsetDID_333=0, OutVarName_333=DID_333, DataType_DID_334=int8, ResolDID_334=1, OffsetDID_334=0, OutVarName_334=DID_334, DataType_DID_335=int8, ResolDID_335=1, OffsetDID_335=0, OutVarName_335=DID_335, DataType_DID_336=int8, ResolDID_336=1, OffsetDID_336=0, OutVarName_336=DID_336, DataType_DID_337=int8, ResolDID_337=1, OffsetDID_337=0, OutVarName_337=DID_337, DataType_DID_338=int8, ResolDID_338=1, OffsetDID_338=0, OutVarName_338=DID_338, DataType_DID_339=int8, ResolDID_339=1, OffsetDID_339=0, OutVarName_339=DID_339, DataType_DID_340=int8, ResolDID_340=1, OffsetDID_340=0, OutVarName_340=DID_340, DataType_DID_341=int8, ResolDID_341=1, OffsetDID_341=0, OutVarName_341=DID_341, DataType_DID_342=int8, ResolDID_342=1, OffsetDID_342=0, OutVarName_342=DID_342, DataType_DID_343=int8, ResolDID_343=1, OffsetDID_343=0, OutVarName_343=DID_343, DataType_DID_344=int8, ResolDID_344=1, OffsetDID_344=0, OutVarName_344=DID_344, DataType_DID_345=int8, ResolDID_345=1, OffsetDID_345=0, OutVarName_345=DID_345, DataType_DID_346=int8, ResolDID_346=1, OffsetDID_346=0, OutVarName_346=DID_346, DataType_DID_347=int8, ResolDID_347=1, OffsetDID_347=0, OutVarName_347=DID_347, DataType_DID_348=int8, ResolDID_348=1, OffsetDID_348=0, OutVarName_348=DID_348, DataType_DID_349=int8, ResolDID_349=1, OffsetDID_349=0, OutVarName_349=DID_349, DataType_DID_350=int8, ResolDID_350=1, OffsetDID_350=0, OutVarName_350=DID_350, DataType_DID_351=int8, ResolDID_351=1, OffsetDID_351=0, OutVarName_351=DID_351, DataType_DID_352=int8, ResolDID_352=1, OffsetDID_352=0, OutVarName_352=DID_352, DataType_DID_353=int8, ResolDID_353=1, OffsetDID_353=0, OutVarName_353=DID_353, DataType_DID_354=int8, ResolDID_354=1, OffsetDID_354=0, OutVarName_354=DID_354, DataType_DID_355=int8, ResolDID_355=1, OffsetDID_355=0, OutVarName_355=DID_355, DataType_DID_356=int8, ResolDID_356=1, OffsetDID_356=0, OutVarName_356=DID_356, DataType_DID_357=int8, ResolDID_357=1, OffsetDID_357=0, OutVarName_357=DID_357, DataType_DID_358=int8, ResolDID_358=1, OffsetDID_358=0, OutVarName_358=DID_358, DataType_DID_359=int8, ResolDID_359=1, OffsetDID_359=0, OutVarName_359=DID_359, DataType_DID_360=int8, ResolDID_360=1, OffsetDID_360=0, OutVarName_360=DID_360, DataType_DID_361=int8, ResolDID_361=1, OffsetDID_361=0, OutVarName_361=DID_361, DataType_DID_362=int8, ResolDID_362=1, OffsetDID_362=0, OutVarName_362=DID_362, DataType_DID_363=int8, ResolDID_363=1, OffsetDID_363=0, OutVarName_363=DID_363, DataType_DID_364=int8, ResolDID_364=1, OffsetDID_364=0, OutVarName_364=DID_364, DataType_DID_365=int8, ResolDID_365=1, OffsetDID_365=0, OutVarName_365=DID_365, DataType_DID_366=int8, ResolDID_366=1, OffsetDID_366=0, OutVarName_366=DID_366, DataType_DID_367=int8, ResolDID_367=1, OffsetDID_367=0, OutVarName_367=DID_367, DataType_DID_368=int8, ResolDID_368=1, OffsetDID_368=0, OutVarName_368=DID_368, DataType_DID_369=int8, ResolDID_369=1, OffsetDID_369=0, OutVarName_369=DID_369, DataType_DID_370=int8, ResolDID_370=1, OffsetDID_370=0, OutVarName_370=DID_370, DataType_DID_371=int8, ResolDID_371=1, OffsetDID_371=0, OutVarName_371=DID_371, DataType_DID_372=int8, ResolDID_372=1, OffsetDID_372=0, OutVarName_372=DID_372, DataType_DID_373=int8, ResolDID_373=1, OffsetDID_373=0, OutVarName_373=DID_373, DataType_DID_374=int8, ResolDID_374=1, OffsetDID_374=0, OutVarName_374=DID_374, DataType_DID_375=int8, ResolDID_375=1, OffsetDID_375=0, OutVarName_375=DID_375, DataType_DID_376=int8, ResolDID_376=1, OffsetDID_376=0, OutVarName_376=DID_376, DataType_DID_377=int8, ResolDID_377=1, OffsetDID_377=0, OutVarName_377=DID_377, DataType_DID_378=int8, ResolDID_378=1, OffsetDID_378=0, OutVarName_378=DID_378, DataType_DID_379=int8, ResolDID_379=1, OffsetDID_379=0, OutVarName_379=DID_379, DataType_DID_380=int8, ResolDID_380=1, OffsetDID_380=0, OutVarName_380=DID_380, DataType_DID_381=int8, ResolDID_381=1, OffsetDID_381=0, OutVarName_381=DID_381, DataType_DID_382=int8, ResolDID_382=1, OffsetDID_382=0, OutVarName_382=DID_382, DataType_DID_383=int8, ResolDID_383=1, OffsetDID_383=0, OutVarName_383=DID_383, DataType_DID_384=int8, ResolDID_384=1, OffsetDID_384=0, OutVarName_384=DID_384, DataType_DID_385=int8, ResolDID_385=1, OffsetDID_385=0, OutVarName_385=DID_385, DataType_DID_386=int8, ResolDID_386=1, OffsetDID_386=0, OutVarName_386=DID_386, DataType_DID_387=int8, ResolDID_387=1, OffsetDID_387=0, OutVarName_387=DID_387, DataType_DID_388=int8, ResolDID_388=1, OffsetDID_388=0, OutVarName_388=DID_388, DataType_DID_389=int8, ResolDID_389=1, OffsetDID_389=0, OutVarName_389=DID_389, DataType_DID_390=int8, ResolDID_390=1, OffsetDID_390=0, OutVarName_390=DID_390, DataType_DID_391=int8, ResolDID_391=1, OffsetDID_391=0, OutVarName_391=DID_391, DataType_DID_392=int8, ResolDID_392=1, OffsetDID_392=0, OutVarName_392=DID_392, DataType_DID_393=int8, ResolDID_393=1, OffsetDID_393=0, OutVarName_393=DID_393, DataType_DID_394=int8, ResolDID_394=1, OffsetDID_394=0, OutVarName_394=DID_394, DataType_DID_395=int8, ResolDID_395=1, OffsetDID_395=0, OutVarName_395=DID_395, DataType_DID_396=int8, ResolDID_396=1, OffsetDID_396=0, OutVarName_396=DID_396, DataType_DID_397=int8, ResolDID_397=1, OffsetDID_397=0, OutVarName_397=DID_397, DataType_DID_398=int8, ResolDID_398=1, OffsetDID_398=0, OutVarName_398=DID_398, DataType_DID_399=int8, ResolDID_399=1, OffsetDID_399=0, OutVarName_399=DID_399, DataType_DID_400=int8, ResolDID_400=1, OffsetDID_400=0, OutVarName_400=DID_400}
      mask prompts: ConfigManagement "Configuration Management"; DIDAbstract "DID Abstract"; NumDIDVar "Number of DID Variables"; DataType_DID_1 "DID Monitoring DataType"; ResolDID_1 "Resolution"; OffsetDID_1 "Offset"; OutVarName_1 "Output Variable"; DataType_DID_2 "DID Monitoring DataType"; ResolDID_2 "Resolution"; OffsetDID_2 "Offset"; OutVarName_2 "Output Variable"; DataType_DID_3 "DID Monitoring DataType"; ResolDID_3 "Resolution"; OffsetDID_3 "Offset"; OutVarName_3 "Output Variable"; DataType_DID_4 "DID Monitoring DataType"; ResolDID_4 "Resolution"; OffsetDID_4 "Offset"; OutVarName_4 "Output Variable"; DataType_DID_5 "DID Monitoring DataType"; ResolDID_5 "Resolution"; OffsetDID_5 "Offset"; OutVarName_5 "Output Variable"; DataType_DID_6 "DID Monitoring DataType"; ResolDID_6 "Resolution"; OffsetDID_6 "Offset"; OutVarName_6 "Output Variable"; DataType_DID_7 "DID Monitoring DataType"; ResolDID_7 "Resolution"; OffsetDID_7 "Offset"; OutVarName_7 "Output Variable"; DataType_DID_8 "DID Monitoring DataType"; ResolDID_8 "Resolution"; OffsetDID_8 "Offset"; OutVarName_8 "Output Variable"; DataType_DID_9 "DID Monitoring DataType"; ResolDID_9 "Resolution"; OffsetDID_9 "Offset"; OutVarName_9 "Output Variable"; DataType_DID_10 "DID Monitoring DataType"; ResolDID_10 "Resolution"; OffsetDID_10 "Offset"; OutVarName_10 "Output Variable"; DataType_DID_11 "DID Monitoring DataType"; ResolDID_11 "Resolution"; OffsetDID_11 "Offset"; OutVarName_11 "Output Variable"; DataType_DID_12 "DID Monitoring DataType"; ResolDID_12 "Resolution"; OffsetDID_12 "Offset"; OutVarName_12 "Output Variable"; DataType_DID_13 "DID Monitoring DataType"; ResolDID_13 "Resolution"; OffsetDID_13 "Offset"; OutVarName_13 "Output Variable"; DataType_DID_14 "DID Monitoring DataType"; ResolDID_14 "Resolution"; OffsetDID_14 "Offset"; OutVarName_14 "Output Variable"; DataType_DID_15 "DID Monitoring DataType"; ResolDID_15 "Resolution"; OffsetDID_15 "Offset"; OutVarName_15 "Output Variable"; DataType_DID_16 "DID Monitoring DataType"; ResolDID_16 "Resolution"; OffsetDID_16 "Offset"; OutVarName_16 "Output Variable"; DataType_DID_17 "DID Monitoring DataType"; ResolDID_17 "Resolution"; OffsetDID_17 "Offset"; OutVarName_17 "Output Variable"; DataType_DID_18 "DID Monitoring DataType"; ResolDID_18 "Resolution"; OffsetDID_18 "Offset"; OutVarName_18 "Output Variable"; DataType_DID_19 "DID Monitoring DataType"; ResolDID_19 "Resolution"; OffsetDID_19 "Offset"; OutVarName_19 "Output Variable"; DataType_DID_20 "DID Monitoring DataType"; ResolDID_20 "Resolution"; OffsetDID_20 "Offset"; OutVarName_20 "Output Variable"; DataType_DID_21 "DID Monitoring DataType"; ResolDID_21 "Resolution"; OffsetDID_21 "Offset"; OutVarName_21 "Output Variable"; DataType_DID_22 "DID Monitoring DataType"; ResolDID_22 "Resolution"; OffsetDID_22 "Offset"; OutVarName_22 "Output Variable"; DataType_DID_23 "DID Monitoring DataType"; ResolDID_23 "Resolution"; OffsetDID_23 "Offset"; OutVarName_23 "Output Variable"; DataType_DID_24 "DID Monitoring DataType"; ResolDID_24 "Resolution"; OffsetDID_24 "Offset"; OutVarName_24 "Output Variable"; DataType_DID_25 "DID Monitoring DataType"; ResolDID_25 "Resolution"; OffsetDID_25 "Offset"; OutVarName_25 "Output Variable"; DataType_DID_26 "DID Monitoring DataType"; ResolDID_26 "Resolution"; OffsetDID_26 "Offset"; OutVarName_26 "Output Variable"; DataType_DID_27 "DID Monitoring DataType"; ResolDID_27 "Resolution"; OffsetDID_27 "Offset"; OutVarName_27 "Output Variable"; DataType_DID_28 "DID Monitoring DataType"; ResolDID_28 "Resolution"; OffsetDID_28 "Offset"; OutVarName_28 "Output Variable"; DataType_DID_29 "DID Monitoring DataType"; ResolDID_29 "Resolution"; OffsetDID_29 "Offset"; OutVarName_29 "Output Variable"; DataType_DID_30 "DID Monitoring DataType"; ResolDID_30 "Resolution"; OffsetDID_30 "Offset"; OutVarName_30 "Output Variable"; DataType_DID_31 "DID Monitoring DataType"; ResolDID_31 "Resolution"; OffsetDID_31 "Offset"; OutVarName_31 "Output Variable"; DataType_DID_32 "DID Monitoring DataType"; ResolDID_32 "Resolution"; OffsetDID_32 "Offset"; OutVarName_32 "Output Variable"; DataType_DID_33 "DID Monitoring DataType"; ResolDID_33 "Resolution"; OffsetDID_33 "Offset"; OutVarName_33 "Output Variable"; DataType_DID_34 "DID Monitoring DataType"; ResolDID_34 "Resolution"; OffsetDID_34 "Offset"; OutVarName_34 "Output Variable"; DataType_DID_35 "DID Monitoring DataType"; ResolDID_35 "Resolution"; OffsetDID_35 "Offset"; OutVarName_35 "Output Variable"; DataType_DID_36 "DID Monitoring DataType"; ResolDID_36 "Resolution"; OffsetDID_36 "Offset"; OutVarName_36 "Output Variable"; DataType_DID_37 "DID Monitoring DataType"; ResolDID_37 "Resolution"; OffsetDID_37 "Offset"; OutVarName_37 "Output Variable"; DataType_DID_38 "DID Monitoring DataType"; ResolDID_38 "Resolution"; OffsetDID_38 "Offset"; OutVarName_38 "Output Variable"; DataType_DID_39 "DID Monitoring DataType"; ResolDID_39 "Resolution"; OffsetDID_39 "Offset"; OutVarName_39 "Output Variable"; DataType_DID_40 "DID Monitoring DataType"; ResolDID_40 "Resolution"; OffsetDID_40 "Offset"; OutVarName_40 "Output Variable"; DataType_DID_41 "DID Monitoring DataType"; ResolDID_41 "Resolution"; OffsetDID_41 "Offset"; OutVarName_41 "Output Variable"; DataType_DID_42 "DID Monitoring DataType"; ResolDID_42 "Resolution"; OffsetDID_42 "Offset"; OutVarName_42 "Output Variable"; DataType_DID_43 "DID Monitoring DataType"; ResolDID_43 "Resolution"; OffsetDID_43 "Offset"; OutVarName_43 "Output Variable"; DataType_DID_44 "DID Monitoring DataType"; ResolDID_44 "Resolution"; OffsetDID_44 "Offset"; OutVarName_44 "Output Variable"; DataType_DID_45 "DID Monitoring DataType"; ResolDID_45 "Resolution"; OffsetDID_45 "Offset"; OutVarName_45 "Output Variable"; DataType_DID_46 "DID Monitoring DataType"; ResolDID_46 "Resolution"; OffsetDID_46 "Offset"; OutVarName_46 "Output Variable"; DataType_DID_47 "DID Monitoring DataType"; ResolDID_47 "Resolution"; OffsetDID_47 "Offset"; OutVarName_47 "Output Variable"; DataType_DID_48 "DID Monitoring DataType"; ResolDID_48 "Resolution"; OffsetDID_48 "Offset"; OutVarName_48 "Output Variable"; DataType_DID_49 "DID Monitoring DataType"; ResolDID_49 "Resolution"; OffsetDID_49 "Offset"; OutVarName_49 "Output Variable"; DataType_DID_50 "DID Monitoring DataType"; ResolDID_50 "Resolution"; OffsetDID_50 "Offset"; OutVarName_50 "Output Variable"; DataType_DID_51 "DID Monitoring DataType"; ResolDID_51 "Resolution"; OffsetDID_51 "Offset"; OutVarName_51 "Output Variable"; DataType_DID_52 "DID Monitoring DataType"; ResolDID_52 "Resolution"; OffsetDID_52 "Offset"; OutVarName_52 "Output Variable"; DataType_DID_53 "DID Monitoring DataType"; ResolDID_53 "Resolution"; OffsetDID_53 "Offset"; OutVarName_53 "Output Variable"; DataType_DID_54 "DID Monitoring DataType"; ResolDID_54 "Resolution"; OffsetDID_54 "Offset"; OutVarName_54 "Output Variable"; DataType_DID_55 "DID Monitoring DataType"; ResolDID_55 "Resolution"; OffsetDID_55 "Offset"; OutVarName_55 "Output Variable"; DataType_DID_56 "DID Monitoring DataType"; ResolDID_56 "Resolution"; OffsetDID_56 "Offset"; OutVarName_56 "Output Variable"; DataType_DID_57 "DID Monitoring DataType"; ResolDID_57 "Resolution"; OffsetDID_57 "Offset"; OutVarName_57 "Output Variable"; DataType_DID_58 "DID Monitoring DataType"; ResolDID_58 "Resolution"; OffsetDID_58 "Offset"; OutVarName_58 "Output Variable"; DataType_DID_59 "DID Monitoring DataType"; ResolDID_59 "Resolution"; OffsetDID_59 "Offset"; OutVarName_59 "Output Variable"; DataType_DID_60 "DID Monitoring DataType"; ResolDID_60 "Resolution"; OffsetDID_60 "Offset"; OutVarName_60 "Output Variable"; DataType_DID_61 "DID Monitoring DataType"; ResolDID_61 "Resolution"; OffsetDID_61 "Offset"; OutVarName_61 "Output Variable"; DataType_DID_62 "DID Monitoring DataType"; ResolDID_62 "Resolution"; OffsetDID_62 "Offset"; OutVarName_62 "Output Variable"; DataType_DID_63 "DID Monitoring DataType"; ResolDID_63 "Resolution"; OffsetDID_63 "Offset"; OutVarName_63 "Output Variable"; DataType_DID_64 "DID Monitoring DataType"; ResolDID_64 "Resolution"; OffsetDID_64 "Offset"; OutVarName_64 "Output Variable"; DataType_DID_65 "DID Monitoring DataType"; ResolDID_65 "Resolution"; OffsetDID_65 "Offset"; OutVarName_65 "Output Variable"; DataType_DID_66 "DID Monitoring DataType"; ResolDID_66 "Resolution"; OffsetDID_66 "Offset"; OutVarName_66 "Output Variable"; DataType_DID_67 "DID Monitoring DataType"; ResolDID_67 "Resolution"; OffsetDID_67 "Offset"; OutVarName_67 "Output Variable"; DataType_DID_68 "DID Monitoring DataType"; ResolDID_68 "Resolution"; OffsetDID_68 "Offset"; OutVarName_68 "Output Variable"; DataType_DID_69 "DID Monitoring DataType"; ResolDID_69 "Resolution"; OffsetDID_69 "Offset"; OutVarName_69 "Output Variable"; DataType_DID_70 "DID Monitoring DataType"; ResolDID_70 "Resolution"; OffsetDID_70 "Offset"; OutVarName_70 "Output Variable"; DataType_DID_71 "DID Monitoring DataType"; ResolDID_71 "Resolution"; OffsetDID_71 "Offset"; OutVarName_71 "Output Variable"; DataType_DID_72 "DID Monitoring DataType"; ResolDID_72 "Resolution"; OffsetDID_72 "Offset"; OutVarName_72 "Output Variable"; DataType_DID_73 "DID Monitoring DataType"; ResolDID_73 "Resolution"; OffsetDID_73 "Offset"; OutVarName_73 "Output Variable"; DataType_DID_74 "DID Monitoring DataType"; ResolDID_74 "Resolution"; OffsetDID_74 "Offset"; OutVarName_74 "Output Variable"; DataType_DID_75 "DID Monitoring DataType"; ResolDID_75 "Resolution"; OffsetDID_75 "Offset"; OutVarName_75 "Output Variable"; DataType_DID_76 "DID Monitoring DataType"; ResolDID_76 "Resolution"; OffsetDID_76 "Offset"; OutVarName_76 "Output Variable"; DataType_DID_77 "DID Monitoring DataType"; ResolDID_77 "Resolution"; OffsetDID_77 "Offset"; OutVarName_77 "Output Variable"; DataType_DID_78 "DID Monitoring DataType"; ResolDID_78 "Resolution"; OffsetDID_78 "Offset"; OutVarName_78 "Output Variable"; DataType_DID_79 "DID Monitoring DataType"; ResolDID_79 "Resolution"; OffsetDID_79 "Offset"; OutVarName_79 "Output Variable"; DataType_DID_80 "DID Monitoring DataType"; ResolDID_80 "Resolution"; OffsetDID_80 "Offset"; OutVarName_80 "Output Variable"; DataType_DID_81 "DID Monitoring DataType"; ResolDID_81 "Resolution"; OffsetDID_81 "Offset"; OutVarName_81 "Output Variable"; DataType_DID_82 "DID Monitoring DataType"; ResolDID_82 "Resolution"; OffsetDID_82 "Offset"; OutVarName_82 "Output Variable"; DataType_DID_83 "DID Monitoring DataType"; ResolDID_83 "Resolution"; OffsetDID_83 "Offset"; OutVarName_83 "Output Variable"; DataType_DID_84 "DID Monitoring DataType"; ResolDID_84 "Resolution"; OffsetDID_84 "Offset"; OutVarName_84 "Output Variable"; DataType_DID_85 "DID Monitoring DataType"; ResolDID_85 "Resolution"; OffsetDID_85 "Offset"; OutVarName_85 "Output Variable"; DataType_DID_86 "DID Monitoring DataType"; ResolDID_86 "Resolution"; OffsetDID_86 "Offset"; OutVarName_86 "Output Variable"; DataType_DID_87 "DID Monitoring DataType"; ResolDID_87 "Resolution"; OffsetDID_87 "Offset"; OutVarName_87 "Output Variable"; DataType_DID_88 "DID Monitoring DataType"; ResolDID_88 "Resolution"; OffsetDID_88 "Offset"; OutVarName_88 "Output Variable"; DataType_DID_89 "DID Monitoring DataType"; ResolDID_89 "Resolution"; OffsetDID_89 "Offset"; OutVarName_89 "Output Variable"; DataType_DID_90 "DID Monitoring DataType"; ResolDID_90 "Resolution"; OffsetDID_90 "Offset"; OutVarName_90 "Output Variable"; DataType_DID_91 "DID Monitoring DataType"; ResolDID_91 "Resolution"; OffsetDID_91 "Offset"; OutVarName_91 "Output Variable"; DataType_DID_92 "DID Monitoring DataType"; ResolDID_92 "Resolution"; OffsetDID_92 "Offset"; OutVarName_92 "Output Variable"; DataType_DID_93 "DID Monitoring DataType"; ResolDID_93 "Resolution"; OffsetDID_93 "Offset"; OutVarName_93 "Output Variable"; DataType_DID_94 "DID Monitoring DataType"; ResolDID_94 "Resolution"; OffsetDID_94 "Offset"; OutVarName_94 "Output Variable"; DataType_DID_95 "DID Monitoring DataType"; ResolDID_95 "Resolution"; OffsetDID_95 "Offset"; OutVarName_95 "Output Variable"; DataType_DID_96 "DID Monitoring DataType"; ResolDID_96 "Resolution"; OffsetDID_96 "Offset"; OutVarName_96 "Output Variable"; DataType_DID_97 "DID Monitoring DataType"; ResolDID_97 "Resolution"; OffsetDID_97 "Offset"; OutVarName_97 "Output Variable"; DataType_DID_98 "DID Monitoring DataType"; ResolDID_98 "Resolution"; OffsetDID_98 "Offset"; OutVarName_98 "Output Variable"; DataType_DID_99 "DID Monitoring DataType"; ResolDID_99 "Resolution"; OffsetDID_99 "Offset"; OutVarName_99 "Output Variable"; DataType_DID_100 "DID Monitoring DataType"; ResolDID_100 "Resolution"; OffsetDID_100 "Offset"; OutVarName_100 "Output Variable"; DataType_DID_101 "DID Monitoring DataType"; ResolDID_101 "Resolution"; OffsetDID_101 "Offset"; OutVarName_101 "Output Variable"; DataType_DID_102 "DID Monitoring DataType"; ResolDID_102 "Resolution"; OffsetDID_102 "Offset"; OutVarName_102 "Output Variable"; DataType_DID_103 "DID Monitoring DataType"; ResolDID_103 "Resolution"; OffsetDID_103 "Offset"; OutVarName_103 "Output Variable"; DataType_DID_104 "DID Monitoring DataType"; ResolDID_104 "Resolution"; OffsetDID_104 "Offset"; OutVarName_104 "Output Variable"; DataType_DID_105 "DID Monitoring DataType"; ResolDID_105 "Resolution"; OffsetDID_105 "Offset"; OutVarName_105 "Output Variable"; DataType_DID_106 "DID Monitoring DataType"; ResolDID_106 "Resolution"; OffsetDID_106 "Offset"; OutVarName_106 "Output Variable"; DataType_DID_107 "DID Monitoring DataType"; ResolDID_107 "Resolution"; OffsetDID_107 "Offset"; OutVarName_107 "Output Variable"; DataType_DID_108 "DID Monitoring DataType"; ResolDID_108 "Resolution"; OffsetDID_108 "Offset"; OutVarName_108 "Output Variable"; DataType_DID_109 "DID Monitoring DataType"; ResolDID_109 "Resolution"; OffsetDID_109 "Offset"; OutVarName_109 "Output Variable"; DataType_DID_110 "DID Monitoring DataType"; ResolDID_110 "Resolution"; OffsetDID_110 "Offset"; OutVarName_110 "Output Variable"; DataType_DID_111 "DID Monitoring DataType"; ResolDID_111 "Resolution"; OffsetDID_111 "Offset"; OutVarName_111 "Output Variable"; DataType_DID_112 "DID Monitoring DataType"; ResolDID_112 "Resolution"; OffsetDID_112 "Offset"; OutVarName_112 "Output Variable"; DataType_DID_113 "DID Monitoring DataType"; ResolDID_113 "Resolution"; OffsetDID_113 "Offset"; OutVarName_113 "Output Variable"; DataType_DID_114 "DID Monitoring DataType"; ResolDID_114 "Resolution"; OffsetDID_114 "Offset"; OutVarName_114 "Output Variable"; DataType_DID_115 "DID Monitoring DataType"; ResolDID_115 "Resolution"; OffsetDID_115 "Offset"; OutVarName_115 "Output Variable"; DataType_DID_116 "DID Monitoring DataType"; ResolDID_116 "Resolution"; OffsetDID_116 "Offset"; OutVarName_116 "Output Variable"; DataType_DID_117 "DID Monitoring DataType"; ResolDID_117 "Resolution"; OffsetDID_117 "Offset"; OutVarName_117 "Output Variable"; DataType_DID_118 "DID Monitoring DataType"; ResolDID_118 "Resolution"; OffsetDID_118 "Offset"; OutVarName_118 "Output Variable"; DataType_DID_119 "DID Monitoring DataType"; ResolDID_119 "Resolution"; OffsetDID_119 "Offset"; OutVarName_119 "Output Variable"; DataType_DID_120 "DID Monitoring DataType"; ResolDID_120 "Resolution"; OffsetDID_120 "Offset"; OutVarName_120 "Output Variable"; DataType_DID_121 "DID Monitoring DataType"; ResolDID_121 "Resolution"; OffsetDID_121 "Offset"; OutVarName_121 "Output Variable"; DataType_DID_122 "DID Monitoring DataType"; ResolDID_122 "Resolution"; OffsetDID_122 "Offset"; OutVarName_122 "Output Variable"; DataType_DID_123 "DID Monitoring DataType"; ResolDID_123 "Resolution"; OffsetDID_123 "Offset"; OutVarName_123 "Output Variable"; DataType_DID_124 "DID Monitoring DataType"; ResolDID_124 "Resolution"; OffsetDID_124 "Offset"; OutVarName_124 "Output Variable"; DataType_DID_125 "DID Monitoring DataType"; ResolDID_125 "Resolution"; OffsetDID_125 "Offset"; OutVarName_125 "Output Variable"; DataType_DID_126 "DID Monitoring DataType"; ResolDID_126 "Resolution"; OffsetDID_126 "Offset"; OutVarName_126 "Output Variable"; DataType_DID_127 "DID Monitoring DataType"; ResolDID_127 "Resolution"; OffsetDID_127 "Offset"; OutVarName_127 "Output Variable"; DataType_DID_128 "DID Monitoring DataType"; ResolDID_128 "Resolution"; OffsetDID_128 "Offset"; OutVarName_128 "Output Variable"; DataType_DID_129 "DID Monitoring DataType"; ResolDID_129 "Resolution"; OffsetDID_129 "Offset"; OutVarName_129 "Output Variable"; DataType_DID_130 "DID Monitoring DataType"; ResolDID_130 "Resolution"; OffsetDID_130 "Offset"; OutVarName_130 "Output Variable"; DataType_DID_131 "DID Monitoring DataType"; ResolDID_131 "Resolution"; OffsetDID_131 "Offset"; OutVarName_131 "Output Variable"; DataType_DID_132 "DID Monitoring DataType"; ResolDID_132 "Resolution"; OffsetDID_132 "Offset"; OutVarName_132 "Output Variable"; DataType_DID_133 "DID Monitoring DataType"; ResolDID_133 "Resolution"; OffsetDID_133 "Offset"; OutVarName_133 "Output Variable"; DataType_DID_134 "DID Monitoring DataType"; ResolDID_134 "Resolution"; OffsetDID_134 "Offset"; OutVarName_134 "Output Variable"; DataType_DID_135 "DID Monitoring DataType"; ResolDID_135 "Resolution"; OffsetDID_135 "Offset"; OutVarName_135 "Output Variable"; DataType_DID_136 "DID Monitoring DataType"; ResolDID_136 "Resolution"; OffsetDID_136 "Offset"; OutVarName_136 "Output Variable"; DataType_DID_137 "DID Monitoring DataType"; ResolDID_137 "Resolution"; OffsetDID_137 "Offset"; OutVarName_137 "Output Variable"; DataType_DID_138 "DID Monitoring DataType"; ResolDID_138 "Resolution"; OffsetDID_138 "Offset"; OutVarName_138 "Output Variable"; DataType_DID_139 "DID Monitoring DataType"; ResolDID_139 "Resolution"; OffsetDID_139 "Offset"; OutVarName_139 "Output Variable"; DataType_DID_140 "DID Monitoring DataType"; ResolDID_140 "Resolution"; OffsetDID_140 "Offset"; OutVarName_140 "Output Variable"; DataType_DID_141 "DID Monitoring DataType"; ResolDID_141 "Resolution"; OffsetDID_141 "Offset"; OutVarName_141 "Output Variable"; DataType_DID_142 "DID Monitoring DataType"; ResolDID_142 "Resolution"; OffsetDID_142 "Offset"; OutVarName_142 "Output Variable"; DataType_DID_143 "DID Monitoring DataType"; ResolDID_143 "Resolution"; OffsetDID_143 "Offset"; OutVarName_143 "Output Variable"; DataType_DID_144 "DID Monitoring DataType"; ResolDID_144 "Resolution"; OffsetDID_144 "Offset"; OutVarName_144 "Output Variable"; DataType_DID_145 "DID Monitoring DataType"; ResolDID_145 "Resolution"; OffsetDID_145 "Offset"; OutVarName_145 "Output Variable"; DataType_DID_146 "DID Monitoring DataType"; ResolDID_146 "Resolution"; OffsetDID_146 "Offset"; OutVarName_146 "Output Variable"; DataType_DID_147 "DID Monitoring DataType"; ResolDID_147 "Resolution"; OffsetDID_147 "Offset"; OutVarName_147 "Output Variable"; DataType_DID_148 "DID Monitoring DataType"; ResolDID_148 "Resolution"; OffsetDID_148 "Offset"; OutVarName_148 "Output Variable"; DataType_DID_149 "DID Monitoring DataType"; ResolDID_149 "Resolution"; OffsetDID_149 "Offset"; OutVarName_149 "Output Variable"; DataType_DID_150 "DID Monitoring DataType"; ResolDID_150 "Resolution"; OffsetDID_150 "Offset"; OutVarName_150 "Output Variable"; DataType_DID_151 "DID Monitoring DataType"; ResolDID_151 "Resolution"; OffsetDID_151 "Offset"; OutVarName_151 "Output Variable"; DataType_DID_152 "DID Monitoring DataType"; ResolDID_152 "Resolution"; OffsetDID_152 "Offset"; OutVarName_152 "Output Variable"; DataType_DID_153 "DID Monitoring DataType"; ResolDID_153 "Resolution"; OffsetDID_153 "Offset"; OutVarName_153 "Output Variable"; DataType_DID_154 "DID Monitoring DataType"; ResolDID_154 "Resolution"; OffsetDID_154 "Offset"; OutVarName_154 "Output Variable"; DataType_DID_155 "DID Monitoring DataType"; ResolDID_155 "Resolution"; OffsetDID_155 "Offset"; OutVarName_155 "Output Variable"; DataType_DID_156 "DID Monitoring DataType"; ResolDID_156 "Resolution"; OffsetDID_156 "Offset"; OutVarName_156 "Output Variable"; DataType_DID_157 "DID Monitoring DataType"; ResolDID_157 "Resolution"; OffsetDID_157 "Offset"; OutVarName_157 "Output Variable"; DataType_DID_158 "DID Monitoring DataType"; ResolDID_158 "Resolution"; OffsetDID_158 "Offset"; OutVarName_158 "Output Variable"; DataType_DID_159 "DID Monitoring DataType"; ResolDID_159 "Resolution"; OffsetDID_159 "Offset"; OutVarName_159 "Output Variable"; DataType_DID_160 "DID Monitoring DataType"; ResolDID_160 "Resolution"; OffsetDID_160 "Offset"; OutVarName_160 "Output Variable"; DataType_DID_161 "DID Monitoring DataType"; ResolDID_161 "Resolution"; OffsetDID_161 "Offset"; OutVarName_161 "Output Variable"; DataType_DID_162 "DID Monitoring DataType"; ResolDID_162 "Resolution"; OffsetDID_162 "Offset"; OutVarName_162 "Output Variable"; DataType_DID_163 "DID Monitoring DataType"; ResolDID_163 "Resolution"; OffsetDID_163 "Offset"; OutVarName_163 "Output Variable"; DataType_DID_164 "DID Monitoring DataType"; ResolDID_164 "Resolution"; OffsetDID_164 "Offset"; OutVarName_164 "Output Variable"; DataType_DID_165 "DID Monitoring DataType"; ResolDID_165 "Resolution"; OffsetDID_165 "Offset"; OutVarName_165 "Output Variable"; DataType_DID_166 "DID Monitoring DataType"; ResolDID_166 "Resolution"; OffsetDID_166 "Offset"; OutVarName_166 "Output Variable"; DataType_DID_167 "DID Monitoring DataType"; ResolDID_167 "Resolution"; OffsetDID_167 "Offset"; OutVarName_167 "Output Variable"; DataType_DID_168 "DID Monitoring DataType"; ResolDID_168 "Resolution"; OffsetDID_168 "Offset"; OutVarName_168 "Output Variable"; DataType_DID_169 "DID Monitoring DataType"; ResolDID_169 "Resolution"; OffsetDID_169 "Offset"; OutVarName_169 "Output Variable"; DataType_DID_170 "DID Monitoring DataType"; ResolDID_170 "Resolution"; OffsetDID_170 "Offset"; OutVarName_170 "Output Variable"; DataType_DID_171 "DID Monitoring DataType"; ResolDID_171 "Resolution"; OffsetDID_171 "Offset"; OutVarName_171 "Output Variable"; DataType_DID_172 "DID Monitoring DataType"; ResolDID_172 "Resolution"; OffsetDID_172 "Offset"; OutVarName_172 "Output Variable"; DataType_DID_173 "DID Monitoring DataType"; ResolDID_173 "Resolution"; OffsetDID_173 "Offset"; OutVarName_173 "Output Variable"; DataType_DID_174 "DID Monitoring DataType"; ResolDID_174 "Resolution"; OffsetDID_174 "Offset"; OutVarName_174 "Output Variable"; DataType_DID_175 "DID Monitoring DataType"; ResolDID_175 "Resolution"; OffsetDID_175 "Offset"; OutVarName_175 "Output Variable"; DataType_DID_176 "DID Monitoring DataType"; ResolDID_176 "Resolution"; OffsetDID_176 "Offset"; OutVarName_176 "Output Variable"; DataType_DID_177 "DID Monitoring DataType"; ResolDID_177 "Resolution"; OffsetDID_177 "Offset"; OutVarName_177 "Output Variable"; DataType_DID_178 "DID Monitoring DataType"; ResolDID_178 "Resolution"; OffsetDID_178 "Offset"; OutVarName_178 "Output Variable"; DataType_DID_179 "DID Monitoring DataType"; ResolDID_179 "Resolution"; OffsetDID_179 "Offset"; OutVarName_179 "Output Variable"; DataType_DID_180 "DID Monitoring DataType"; ResolDID_180 "Resolution"; OffsetDID_180 "Offset"; OutVarName_180 "Output Variable"; DataType_DID_181 "DID Monitoring DataType"; ResolDID_181 "Resolution"; OffsetDID_181 "Offset"; OutVarName_181 "Output Variable"; DataType_DID_182 "DID Monitoring DataType"; ResolDID_182 "Resolution"; OffsetDID_182 "Offset"; OutVarName_182 "Output Variable"; DataType_DID_183 "DID Monitoring DataType"; ResolDID_183 "Resolution"; OffsetDID_183 "Offset"; OutVarName_183 "Output Variable"; DataType_DID_184 "DID Monitoring DataType"; ResolDID_184 "Resolution"; OffsetDID_184 "Offset"; OutVarName_184 "Output Variable"; DataType_DID_185 "DID Monitoring DataType"; ResolDID_185 "Resolution"; OffsetDID_185 "Offset"; OutVarName_185 "Output Variable"; DataType_DID_186 "DID Monitoring DataType"; ResolDID_186 "Resolution"; OffsetDID_186 "Offset"; OutVarName_186 "Output Variable"; DataType_DID_187 "DID Monitoring DataType"; ResolDID_187 "Resolution"; OffsetDID_187 "Offset"; OutVarName_187 "Output Variable"; DataType_DID_188 "DID Monitoring DataType"; ResolDID_188 "Resolution"; OffsetDID_188 "Offset"; OutVarName_188 "Output Variable"; DataType_DID_189 "DID Monitoring DataType"; ResolDID_189 "Resolution"; OffsetDID_189 "Offset"; OutVarName_189 "Output Variable"; DataType_DID_190 "DID Monitoring DataType"; ResolDID_190 "Resolution"; OffsetDID_190 "Offset"; OutVarName_190 "Output Variable"; DataType_DID_191 "DID Monitoring DataType"; ResolDID_191 "Resolution"; OffsetDID_191 "Offset"; OutVarName_191 "Output Variable"; DataType_DID_192 "DID Monitoring DataType"; ResolDID_192 "Resolution"; OffsetDID_192 "Offset"; OutVarName_192 "Output Variable"; DataType_DID_193 "DID Monitoring DataType"; ResolDID_193 "Resolution"; OffsetDID_193 "Offset"; OutVarName_193 "Output Variable"; DataType_DID_194 "DID Monitoring DataType"; ResolDID_194 "Resolution"; OffsetDID_194 "Offset"; OutVarName_194 "Output Variable"; DataType_DID_195 "DID Monitoring DataType"; ResolDID_195 "Resolution"; OffsetDID_195 "Offset"; OutVarName_195 "Output Variable"; DataType_DID_196 "DID Monitoring DataType"; ResolDID_196 "Resolution"; OffsetDID_196 "Offset"; OutVarName_196 "Output Variable"; DataType_DID_197 "DID Monitoring DataType"; ResolDID_197 "Resolution"; OffsetDID_197 "Offset"; OutVarName_197 "Output Variable"; DataType_DID_198 "DID Monitoring DataType"; ResolDID_198 "Resolution"; OffsetDID_198 "Offset"; OutVarName_198 "Output Variable"; DataType_DID_199 "DID Monitoring DataType"; ResolDID_199 "Resolution"; OffsetDID_199 "Offset"; OutVarName_199 "Output Variable"; DataType_DID_200 "DID Monitoring DataType"; ResolDID_200 "Resolution"; OffsetDID_200 "Offset"; OutVarName_200 "Output Variable"; DataType_DID_201 "DID Monitoring DataType"; ResolDID_201 "Resolution"; OffsetDID_201 "Offset"; OutVarName_201 "Output Variable"; DataType_DID_202 "DID Monitoring DataType"; ResolDID_202 "Resolution"; OffsetDID_202 "Offset"; OutVarName_202 "Output Variable"; DataType_DID_203 "DID Monitoring DataType"; ResolDID_203 "Resolution"; OffsetDID_203 "Offset"; OutVarName_203 "Output Variable"; DataType_DID_204 "DID Monitoring DataType"; ResolDID_204 "Resolution"; OffsetDID_204 "Offset"; OutVarName_204 "Output Variable"; DataType_DID_205 "DID Monitoring DataType"; ResolDID_205 "Resolution"; OffsetDID_205 "Offset"; OutVarName_205 "Output Variable"; DataType_DID_206 "DID Monitoring DataType"; ResolDID_206 "Resolution"; OffsetDID_206 "Offset"; OutVarName_206 "Output Variable"; DataType_DID_207 "DID Monitoring DataType"; ResolDID_207 "Resolution"; OffsetDID_207 "Offset"; OutVarName_207 "Output Variable"; DataType_DID_208 "DID Monitoring DataType"; ResolDID_208 "Resolution"; OffsetDID_208 "Offset"; OutVarName_208 "Output Variable"; DataType_DID_209 "DID Monitoring DataType"; ResolDID_209 "Resolution"; OffsetDID_209 "Offset"; OutVarName_209 "Output Variable"; DataType_DID_210 "DID Monitoring DataType"; ResolDID_210 "Resolution"; OffsetDID_210 "Offset"; OutVarName_210 "Output Variable"; DataType_DID_211 "DID Monitoring DataType"; ResolDID_211 "Resolution"; OffsetDID_211 "Offset"; OutVarName_211 "Output Variable"; DataType_DID_212 "DID Monitoring DataType"; ResolDID_212 "Resolution"; OffsetDID_212 "Offset"; OutVarName_212 "Output Variable"; DataType_DID_213 "DID Monitoring DataType"; ResolDID_213 "Resolution"; OffsetDID_213 "Offset"; OutVarName_213 "Output Variable"; DataType_DID_214 "DID Monitoring DataType"; ResolDID_214 "Resolution"; OffsetDID_214 "Offset"; OutVarName_214 "Output Variable"; DataType_DID_215 "DID Monitoring DataType"; ResolDID_215 "Resolution"; OffsetDID_215 "Offset"; OutVarName_215 "Output Variable"; DataType_DID_216 "DID Monitoring DataType"; ResolDID_216 "Resolution"; OffsetDID_216 "Offset"; OutVarName_216 "Output Variable"; DataType_DID_217 "DID Monitoring DataType"; ResolDID_217 "Resolution"; OffsetDID_217 "Offset"; OutVarName_217 "Output Variable"; DataType_DID_218 "DID Monitoring DataType"; ResolDID_218 "Resolution"; OffsetDID_218 "Offset"; OutVarName_218 "Output Variable"; DataType_DID_219 "DID Monitoring DataType"; ResolDID_219 "Resolution"; OffsetDID_219 "Offset"; OutVarName_219 "Output Variable"; DataType_DID_220 "DID Monitoring DataType"; ResolDID_220 "Resolution"; OffsetDID_220 "Offset"; OutVarName_220 "Output Variable"; DataType_DID_221 "DID Monitoring DataType"; ResolDID_221 "Resolution"; OffsetDID_221 "Offset"; OutVarName_221 "Output Variable"; DataType_DID_222 "DID Monitoring DataType"; ResolDID_222 "Resolution"; OffsetDID_222 "Offset"; OutVarName_222 "Output Variable"; DataType_DID_223 "DID Monitoring DataType"; ResolDID_223 "Resolution"; OffsetDID_223 "Offset"; OutVarName_223 "Output Variable"; DataType_DID_224 "DID Monitoring DataType"; ResolDID_224 "Resolution"; OffsetDID_224 "Offset"; OutVarName_224 "Output Variable"; DataType_DID_225 "DID Monitoring DataType"; ResolDID_225 "Resolution"; OffsetDID_225 "Offset"; OutVarName_225 "Output Variable"; DataType_DID_226 "DID Monitoring DataType"; ResolDID_226 "Resolution"; OffsetDID_226 "Offset"; OutVarName_226 "Output Variable"; DataType_DID_227 "DID Monitoring DataType"; ResolDID_227 "Resolution"; OffsetDID_227 "Offset"; OutVarName_227 "Output Variable"; DataType_DID_228 "DID Monitoring DataType"; ResolDID_228 "Resolution"; OffsetDID_228 "Offset"; OutVarName_228 "Output Variable"; DataType_DID_229 "DID Monitoring DataType"; ResolDID_229 "Resolution"; OffsetDID_229 "Offset"; OutVarName_229 "Output Variable"; DataType_DID_230 "DID Monitoring DataType"; ResolDID_230 "Resolution"; OffsetDID_230 "Offset"; OutVarName_230 "Output Variable"; DataType_DID_231 "DID Monitoring DataType"; ResolDID_231 "Resolution"; OffsetDID_231 "Offset"; OutVarName_231 "Output Variable"; DataType_DID_232 "DID Monitoring DataType"; ResolDID_232 "Resolution"; OffsetDID_232 "Offset"; OutVarName_232 "Output Variable"; DataType_DID_233 "DID Monitoring DataType"; ResolDID_233 "Resolution"; OffsetDID_233 "Offset"; OutVarName_233 "Output Variable"; DataType_DID_234 "DID Monitoring DataType"; ResolDID_234 "Resolution"; OffsetDID_234 "Offset"; OutVarName_234 "Output Variable"; DataType_DID_235 "DID Monitoring DataType"; ResolDID_235 "Resolution"; OffsetDID_235 "Offset"; OutVarName_235 "Output Variable"; DataType_DID_236 "DID Monitoring DataType"; ResolDID_236 "Resolution"; OffsetDID_236 "Offset"; OutVarName_236 "Output Variable"; DataType_DID_237 "DID Monitoring DataType"; ResolDID_237 "Resolution"; OffsetDID_237 "Offset"; OutVarName_237 "Output Variable"; DataType_DID_238 "DID Monitoring DataType"; ResolDID_238 "Resolution"; OffsetDID_238 "Offset"; OutVarName_238 "Output Variable"; DataType_DID_239 "DID Monitoring DataType"; ResolDID_239 "Resolution"; OffsetDID_239 "Offset"; OutVarName_239 "Output Variable"; DataType_DID_240 "DID Monitoring DataType"; ResolDID_240 "Resolution"; OffsetDID_240 "Offset"; OutVarName_240 "Output Variable"; DataType_DID_241 "DID Monitoring DataType"; ResolDID_241 "Resolution"; OffsetDID_241 "Offset"; OutVarName_241 "Output Variable"; DataType_DID_242 "DID Monitoring DataType"; ResolDID_242 "Resolution"; OffsetDID_242 "Offset"; OutVarName_242 "Output Variable"; DataType_DID_243 "DID Monitoring DataType"; ResolDID_243 "Resolution"; OffsetDID_243 "Offset"; OutVarName_243 "Output Variable"; DataType_DID_244 "DID Monitoring DataType"; ResolDID_244 "Resolution"; OffsetDID_244 "Offset"; OutVarName_244 "Output Variable"; DataType_DID_245 "DID Monitoring DataType"; ResolDID_245 "Resolution"; OffsetDID_245 "Offset"; OutVarName_245 "Output Variable"; DataType_DID_246 "DID Monitoring DataType"; ResolDID_246 "Resolution"; OffsetDID_246 "Offset"; OutVarName_246 "Output Variable"; DataType_DID_247 "DID Monitoring DataType"; ResolDID_247 "Resolution"; OffsetDID_247 "Offset"; OutVarName_247 "Output Variable"; DataType_DID_248 "DID Monitoring DataType"; ResolDID_248 "Resolution"; OffsetDID_248 "Offset"; OutVarName_248 "Output Variable"; DataType_DID_249 "DID Monitoring DataType"; ResolDID_249 "Resolution"; OffsetDID_249 "Offset"; OutVarName_249 "Output Variable"; DataType_DID_250 "DID Monitoring DataType"; ResolDID_250 "Resolution"; OffsetDID_250 "Offset"; OutVarName_250 "Output Variable"; DataType_DID_251 "DID Monitoring DataType"; ResolDID_251 "Resolution"; OffsetDID_251 "Offset"; OutVarName_251 "Output Variable"; DataType_DID_252 "DID Monitoring DataType"; ResolDID_252 "Resolution"; OffsetDID_252 "Offset"; OutVarName_252 "Output Variable"; DataType_DID_253 "DID Monitoring DataType"; ResolDID_253 "Resolution"; OffsetDID_253 "Offset"; OutVarName_253 "Output Variable"; DataType_DID_254 "DID Monitoring DataType"; ResolDID_254 "Resolution"; OffsetDID_254 "Offset"; OutVarName_254 "Output Variable"; DataType_DID_255 "DID Monitoring DataType"; ResolDID_255 "Resolution"; OffsetDID_255 "Offset"; OutVarName_255 "Output Variable"; DataType_DID_256 "DID Monitoring DataType"; ResolDID_256 "Resolution"; OffsetDID_256 "Offset"; OutVarName_256 "Output Variable"; DataType_DID_257 "DID Monitoring DataType"; ResolDID_257 "Resolution"; OffsetDID_257 "Offset"; OutVarName_257 "Output Variable"; DataType_DID_258 "DID Monitoring DataType"; ResolDID_258 "Resolution"; OffsetDID_258 "Offset"; OutVarName_258 "Output Variable"; DataType_DID_259 "DID Monitoring DataType"; ResolDID_259 "Resolution"; OffsetDID_259 "Offset"; OutVarName_259 "Output Variable"; DataType_DID_260 "DID Monitoring DataType"; ResolDID_260 "Resolution"; OffsetDID_260 "Offset"; OutVarName_260 "Output Variable"; DataType_DID_261 "DID Monitoring DataType"; ResolDID_261 "Resolution"; OffsetDID_261 "Offset"; OutVarName_261 "Output Variable"; DataType_DID_262 "DID Monitoring DataType"; ResolDID_262 "Resolution"; OffsetDID_262 "Offset"; OutVarName_262 "Output Variable"; DataType_DID_263 "DID Monitoring DataType"; ResolDID_263 "Resolution"; OffsetDID_263 "Offset"; OutVarName_263 "Output Variable"; DataType_DID_264 "DID Monitoring DataType"; ResolDID_264 "Resolution"; OffsetDID_264 "Offset"; OutVarName_264 "Output Variable"; DataType_DID_265 "DID Monitoring DataType"; ResolDID_265 "Resolution"; OffsetDID_265 "Offset"; OutVarName_265 "Output Variable"; DataType_DID_266 "DID Monitoring DataType"; ResolDID_266 "Resolution"; OffsetDID_266 "Offset"; OutVarName_266 "Output Variable"; DataType_DID_267 "DID Monitoring DataType"; ResolDID_267 "Resolution"; OffsetDID_267 "Offset"; OutVarName_267 "Output Variable"; DataType_DID_268 "DID Monitoring DataType"; ResolDID_268 "Resolution"; OffsetDID_268 "Offset"; OutVarName_268 "Output Variable"; DataType_DID_269 "DID Monitoring DataType"; ResolDID_269 "Resolution"; OffsetDID_269 "Offset"; OutVarName_269 "Output Variable"; DataType_DID_270 "DID Monitoring DataType"; ResolDID_270 "Resolution"; OffsetDID_270 "Offset"; OutVarName_270 "Output Variable"; DataType_DID_271 "DID Monitoring DataType"; ResolDID_271 "Resolution"; OffsetDID_271 "Offset"; OutVarName_271 "Output Variable"; DataType_DID_272 "DID Monitoring DataType"; ResolDID_272 "Resolution"; OffsetDID_272 "Offset"; OutVarName_272 "Output Variable"; DataType_DID_273 "DID Monitoring DataType"; ResolDID_273 "Resolution"; OffsetDID_273 "Offset"; OutVarName_273 "Output Variable"; DataType_DID_274 "DID Monitoring DataType"; ResolDID_274 "Resolution"; OffsetDID_274 "Offset"; OutVarName_274 "Output Variable"; DataType_DID_275 "DID Monitoring DataType"; ResolDID_275 "Resolution"; OffsetDID_275 "Offset"; OutVarName_275 "Output Variable"; DataType_DID_276 "DID Monitoring DataType"; ResolDID_276 "Resolution"; OffsetDID_276 "Offset"; OutVarName_276 "Output Variable"; DataType_DID_277 "DID Monitoring DataType"; ResolDID_277 "Resolution"; OffsetDID_277 "Offset"; OutVarName_277 "Output Variable"; DataType_DID_278 "DID Monitoring DataType"; ResolDID_278 "Resolution"; OffsetDID_278 "Offset"; OutVarName_278 "Output Variable"; DataType_DID_279 "DID Monitoring DataType"; ResolDID_279 "Resolution"; OffsetDID_279 "Offset"; OutVarName_279 "Output Variable"; DataType_DID_280 "DID Monitoring DataType"; ResolDID_280 "Resolution"; OffsetDID_280 "Offset"; OutVarName_280 "Output Variable"; DataType_DID_281 "DID Monitoring DataType"; ResolDID_281 "Resolution"; OffsetDID_281 "Offset"; OutVarName_281 "Output Variable"; DataType_DID_282 "DID Monitoring DataType"; ResolDID_282 "Resolution"; OffsetDID_282 "Offset"; OutVarName_282 "Output Variable"; DataType_DID_283 "DID Monitoring DataType"; ResolDID_283 "Resolution"; OffsetDID_283 "Offset"; OutVarName_283 "Output Variable"; DataType_DID_284 "DID Monitoring DataType"; ResolDID_284 "Resolution"; OffsetDID_284 "Offset"; OutVarName_284 "Output Variable"; DataType_DID_285 "DID Monitoring DataType"; ResolDID_285 "Resolution"; OffsetDID_285 "Offset"; OutVarName_285 "Output Variable"; DataType_DID_286 "DID Monitoring DataType"; ResolDID_286 "Resolution"; OffsetDID_286 "Offset"; OutVarName_286 "Output Variable"; DataType_DID_287 "DID Monitoring DataType"; ResolDID_287 "Resolution"; OffsetDID_287 "Offset"; OutVarName_287 "Output Variable"; DataType_DID_288 "DID Monitoring DataType"; ResolDID_288 "Resolution"; OffsetDID_288 "Offset"; OutVarName_288 "Output Variable"; DataType_DID_289 "DID Monitoring DataType"; ResolDID_289 "Resolution"; OffsetDID_289 "Offset"; OutVarName_289 "Output Variable"; DataType_DID_290 "DID Monitoring DataType"; ResolDID_290 "Resolution"; OffsetDID_290 "Offset"; OutVarName_290 "Output Variable"; DataType_DID_291 "DID Monitoring DataType"; ResolDID_291 "Resolution"; OffsetDID_291 "Offset"; OutVarName_291 "Output Variable"; DataType_DID_292 "DID Monitoring DataType"; ResolDID_292 "Resolution"; OffsetDID_292 "Offset"; OutVarName_292 "Output Variable"; DataType_DID_293 "DID Monitoring DataType"; ResolDID_293 "Resolution"; OffsetDID_293 "Offset"; OutVarName_293 "Output Variable"; DataType_DID_294 "DID Monitoring DataType"; ResolDID_294 "Resolution"; OffsetDID_294 "Offset"; OutVarName_294 "Output Variable"; DataType_DID_295 "DID Monitoring DataType"; ResolDID_295 "Resolution"; OffsetDID_295 "Offset"; OutVarName_295 "Output Variable"; DataType_DID_296 "DID Monitoring DataType"; ResolDID_296 "Resolution"; OffsetDID_296 "Offset"; OutVarName_296 "Output Variable"; DataType_DID_297 "DID Monitoring DataType"; ResolDID_297 "Resolution"; OffsetDID_297 "Offset"; OutVarName_297 "Output Variable"; DataType_DID_298 "DID Monitoring DataType"; ResolDID_298 "Resolution"; OffsetDID_298 "Offset"; OutVarName_298 "Output Variable"; DataType_DID_299 "DID Monitoring DataType"; ResolDID_299 "Resolution"; OffsetDID_299 "Offset"; OutVarName_299 "Output Variable"; DataType_DID_300 "DID Monitoring DataType"; ResolDID_300 "Resolution"; OffsetDID_300 "Offset"; OutVarName_300 "Output Variable"; DataType_DID_301 "DID Monitoring DataType"; ResolDID_301 "Resolution"; OffsetDID_301 "Offset"; OutVarName_301 "Output Variable"; DataType_DID_302 "DID Monitoring DataType"; ResolDID_302 "Resolution"; OffsetDID_302 "Offset"; OutVarName_302 "Output Variable"; DataType_DID_303 "DID Monitoring DataType"; ResolDID_303 "Resolution"; OffsetDID_303 "Offset"; OutVarName_303 "Output Variable"; DataType_DID_304 "DID Monitoring DataType"; ResolDID_304 "Resolution"; OffsetDID_304 "Offset"; OutVarName_304 "Output Variable"; DataType_DID_305 "DID Monitoring DataType"; ResolDID_305 "Resolution"; OffsetDID_305 "Offset"; OutVarName_305 "Output Variable"; DataType_DID_306 "DID Monitoring DataType"; ResolDID_306 "Resolution"; OffsetDID_306 "Offset"; OutVarName_306 "Output Variable"; DataType_DID_307 "DID Monitoring DataType"; ResolDID_307 "Resolution"; OffsetDID_307 "Offset"; OutVarName_307 "Output Variable"; DataType_DID_308 "DID Monitoring DataType"; ResolDID_308 "Resolution"; OffsetDID_308 "Offset"; OutVarName_308 "Output Variable"; DataType_DID_309 "DID Monitoring DataType"; ResolDID_309 "Resolution"; OffsetDID_309 "Offset"; OutVarName_309 "Output Variable"; DataType_DID_310 "DID Monitoring DataType"; ResolDID_310 "Resolution"; OffsetDID_310 "Offset"; OutVarName_310 "Output Variable"; DataType_DID_311 "DID Monitoring DataType"; ResolDID_311 "Resolution"; OffsetDID_311 "Offset"; OutVarName_311 "Output Variable"; DataType_DID_312 "DID Monitoring DataType"; ResolDID_312 "Resolution"; OffsetDID_312 "Offset"; OutVarName_312 "Output Variable"; DataType_DID_313 "DID Monitoring DataType"; ResolDID_313 "Resolution"; OffsetDID_313 "Offset"; OutVarName_313 "Output Variable"; DataType_DID_314 "DID Monitoring DataType"; ResolDID_314 "Resolution"; OffsetDID_314 "Offset"; OutVarName_314 "Output Variable"; DataType_DID_315 "DID Monitoring DataType"; ResolDID_315 "Resolution"; OffsetDID_315 "Offset"; OutVarName_315 "Output Variable"; DataType_DID_316 "DID Monitoring DataType"; ResolDID_316 "Resolution"; OffsetDID_316 "Offset"; OutVarName_316 "Output Variable"; DataType_DID_317 "DID Monitoring DataType"; ResolDID_317 "Resolution"; OffsetDID_317 "Offset"; OutVarName_317 "Output Variable"; DataType_DID_318 "DID Monitoring DataType"; ResolDID_318 "Resolution"; OffsetDID_318 "Offset"; OutVarName_318 "Output Variable"; DataType_DID_319 "DID Monitoring DataType"; ResolDID_319 "Resolution"; OffsetDID_319 "Offset"; OutVarName_319 "Output Variable"; DataType_DID_320 "DID Monitoring DataType"; ResolDID_320 "Resolution"; OffsetDID_320 "Offset"; OutVarName_320 "Output Variable"; DataType_DID_321 "DID Monitoring DataType"; ResolDID_321 "Resolution"; OffsetDID_321 "Offset"; OutVarName_321 "Output Variable"; DataType_DID_322 "DID Monitoring DataType"; ResolDID_322 "Resolution"; OffsetDID_322 "Offset"; OutVarName_322 "Output Variable"; DataType_DID_323 "DID Monitoring DataType"; ResolDID_323 "Resolution"; OffsetDID_323 "Offset"; OutVarName_323 "Output Variable"; DataType_DID_324 "DID Monitoring DataType"; ResolDID_324 "Resolution"; OffsetDID_324 "Offset"; OutVarName_324 "Output Variable"; DataType_DID_325 "DID Monitoring DataType"; ResolDID_325 "Resolution"; OffsetDID_325 "Offset"; OutVarName_325 "Output Variable"; DataType_DID_326 "DID Monitoring DataType"; ResolDID_326 "Resolution"; OffsetDID_326 "Offset"; OutVarName_326 "Output Variable"; DataType_DID_327 "DID Monitoring DataType"; ResolDID_327 "Resolution"; OffsetDID_327 "Offset"; OutVarName_327 "Output Variable"; DataType_DID_328 "DID Monitoring DataType"; ResolDID_328 "Resolution"; OffsetDID_328 "Offset"; OutVarName_328 "Output Variable"; DataType_DID_329 "DID Monitoring DataType"; ResolDID_329 "Resolution"; OffsetDID_329 "Offset"; OutVarName_329 "Output Variable"; DataType_DID_330 "DID Monitoring DataType"; ResolDID_330 "Resolution"; OffsetDID_330 "Offset"; OutVarName_330 "Output Variable"; DataType_DID_331 "DID Monitoring DataType"; ResolDID_331 "Resolution"; OffsetDID_331 "Offset"; OutVarName_331 "Output Variable"; DataType_DID_332 "DID Monitoring DataType"; ResolDID_332 "Resolution"; OffsetDID_332 "Offset"; OutVarName_332 "Output Variable"; DataType_DID_333 "DID Monitoring DataType"; ResolDID_333 "Resolution"; OffsetDID_333 "Offset"; OutVarName_333 "Output Variable"; DataType_DID_334 "DID Monitoring DataType"; ResolDID_334 "Resolution"; OffsetDID_334 "Offset"; OutVarName_334 "Output Variable"; DataType_DID_335 "DID Monitoring DataType"; ResolDID_335 "Resolution"; OffsetDID_335 "Offset"; OutVarName_335 "Output Variable"; DataType_DID_336 "DID Monitoring DataType"; ResolDID_336 "Resolution"; OffsetDID_336 "Offset"; OutVarName_336 "Output Variable"; DataType_DID_337 "DID Monitoring DataType"; ResolDID_337 "Resolution"; OffsetDID_337 "Offset"; OutVarName_337 "Output Variable"; DataType_DID_338 "DID Monitoring DataType"; ResolDID_338 "Resolution"; OffsetDID_338 "Offset"; OutVarName_338 "Output Variable"; DataType_DID_339 "DID Monitoring DataType"; ResolDID_339 "Resolution"; OffsetDID_339 "Offset"; OutVarName_339 "Output Variable"; DataType_DID_340 "DID Monitoring DataType"; ResolDID_340 "Resolution"; OffsetDID_340 "Offset"; OutVarName_340 "Output Variable"; DataType_DID_341 "DID Monitoring DataType"; ResolDID_341 "Resolution"; OffsetDID_341 "Offset"; OutVarName_341 "Output Variable"; DataType_DID_342 "DID Monitoring DataType"; ResolDID_342 "Resolution"; OffsetDID_342 "Offset"; OutVarName_342 "Output Variable"; DataType_DID_343 "DID Monitoring DataType"; ResolDID_343 "Resolution"; OffsetDID_343 "Offset"; OutVarName_343 "Output Variable"; DataType_DID_344 "DID Monitoring DataType"; ResolDID_344 "Resolution"; OffsetDID_344 "Offset"; OutVarName_344 "Output Variable"; DataType_DID_345 "DID Monitoring DataType"; ResolDID_345 "Resolution"; OffsetDID_345 "Offset"; OutVarName_345 "Output Variable"; DataType_DID_346 "DID Monitoring DataType"; ResolDID_346 "Resolution"; OffsetDID_346 "Offset"; OutVarName_346 "Output Variable"; DataType_DID_347 "DID Monitoring DataType"; ResolDID_347 "Resolution"; OffsetDID_347 "Offset"; OutVarName_347 "Output Variable"; DataType_DID_348 "DID Monitoring DataType"; ResolDID_348 "Resolution"; OffsetDID_348 "Offset"; OutVarName_348 "Output Variable"; DataType_DID_349 "DID Monitoring DataType"; ResolDID_349 "Resolution"; OffsetDID_349 "Offset"; OutVarName_349 "Output Variable"; DataType_DID_350 "DID Monitoring DataType"; ResolDID_350 "Resolution"; OffsetDID_350 "Offset"; OutVarName_350 "Output Variable"; DataType_DID_351 "DID Monitoring DataType"; ResolDID_351 "Resolution"; OffsetDID_351 "Offset"; OutVarName_351 "Output Variable"; DataType_DID_352 "DID Monitoring DataType"; ResolDID_352 "Resolution"; OffsetDID_352 "Offset"; OutVarName_352 "Output Variable"; DataType_DID_353 "DID Monitoring DataType"; ResolDID_353 "Resolution"; OffsetDID_353 "Offset"; OutVarName_353 "Output Variable"; DataType_DID_354 "DID Monitoring DataType"; ResolDID_354 "Resolution"; OffsetDID_354 "Offset"; OutVarName_354 "Output Variable"; DataType_DID_355 "DID Monitoring DataType"; ResolDID_355 "Resolution"; OffsetDID_355 "Offset"; OutVarName_355 "Output Variable"; DataType_DID_356 "DID Monitoring DataType"; ResolDID_356 "Resolution"; OffsetDID_356 "Offset"; OutVarName_356 "Output Variable"; DataType_DID_357 "DID Monitoring DataType"; ResolDID_357 "Resolution"; OffsetDID_357 "Offset"; OutVarName_357 "Output Variable"; DataType_DID_358 "DID Monitoring DataType"; ResolDID_358 "Resolution"; OffsetDID_358 "Offset"; OutVarName_358 "Output Variable"; DataType_DID_359 "DID Monitoring DataType"; ResolDID_359 "Resolution"; OffsetDID_359 "Offset"; OutVarName_359 "Output Variable"; DataType_DID_360 "DID Monitoring DataType"; ResolDID_360 "Resolution"; OffsetDID_360 "Offset"; OutVarName_360 "Output Variable"; DataType_DID_361 "DID Monitoring DataType"; ResolDID_361 "Resolution"; OffsetDID_361 "Offset"; OutVarName_361 "Output Variable"; DataType_DID_362 "DID Monitoring DataType"; ResolDID_362 "Resolution"; OffsetDID_362 "Offset"; OutVarName_362 "Output Variable"; DataType_DID_363 "DID Monitoring DataType"; ResolDID_363 "Resolution"; OffsetDID_363 "Offset"; OutVarName_363 "Output Variable"; DataType_DID_364 "DID Monitoring DataType"; ResolDID_364 "Resolution"; OffsetDID_364 "Offset"; OutVarName_364 "Output Variable"; DataType_DID_365 "DID Monitoring DataType"; ResolDID_365 "Resolution"; OffsetDID_365 "Offset"; OutVarName_365 "Output Variable"; DataType_DID_366 "DID Monitoring DataType"; ResolDID_366 "Resolution"; OffsetDID_366 "Offset"; OutVarName_366 "Output Variable"; DataType_DID_367 "DID Monitoring DataType"; ResolDID_367 "Resolution"; OffsetDID_367 "Offset"; OutVarName_367 "Output Variable"; DataType_DID_368 "DID Monitoring DataType"; ResolDID_368 "Resolution"; OffsetDID_368 "Offset"; OutVarName_368 "Output Variable"; DataType_DID_369 "DID Monitoring DataType"; ResolDID_369 "Resolution"; OffsetDID_369 "Offset"; OutVarName_369 "Output Variable"; DataType_DID_370 "DID Monitoring DataType"; ResolDID_370 "Resolution"; OffsetDID_370 "Offset"; OutVarName_370 "Output Variable"; DataType_DID_371 "DID Monitoring DataType"; ResolDID_371 "Resolution"; OffsetDID_371 "Offset"; OutVarName_371 "Output Variable"; DataType_DID_372 "DID Monitoring DataType"; ResolDID_372 "Resolution"; OffsetDID_372 "Offset"; OutVarName_372 "Output Variable"; DataType_DID_373 "DID Monitoring DataType"; ResolDID_373 "Resolution"; OffsetDID_373 "Offset"; OutVarName_373 "Output Variable"; DataType_DID_374 "DID Monitoring DataType"; ResolDID_374 "Resolution"; OffsetDID_374 "Offset"; OutVarName_374 "Output Variable"; DataType_DID_375 "DID Monitoring DataType"; ResolDID_375 "Resolution"; OffsetDID_375 "Offset"; OutVarName_375 "Output Variable"; DataType_DID_376 "DID Monitoring DataType"; ResolDID_376 "Resolution"; OffsetDID_376 "Offset"; OutVarName_376 "Output Variable"; DataType_DID_377 "DID Monitoring DataType"; ResolDID_377 "Resolution"; OffsetDID_377 "Offset"; OutVarName_377 "Output Variable"; DataType_DID_378 "DID Monitoring DataType"; ResolDID_378 "Resolution"; OffsetDID_378 "Offset"; OutVarName_378 "Output Variable"; DataType_DID_379 "DID Monitoring DataType"; ResolDID_379 "Resolution"; OffsetDID_379 "Offset"; OutVarName_379 "Output Variable"; DataType_DID_380 "DID Monitoring DataType"; ResolDID_380 "Resolution"; OffsetDID_380 "Offset"; OutVarName_380 "Output Variable"; DataType_DID_381 "DID Monitoring DataType"; ResolDID_381 "Resolution"; OffsetDID_381 "Offset"; OutVarName_381 "Output Variable"; DataType_DID_382 "DID Monitoring DataType"; ResolDID_382 "Resolution"; OffsetDID_382 "Offset"; OutVarName_382 "Output Variable"; DataType_DID_383 "DID Monitoring DataType"; ResolDID_383 "Resolution"; OffsetDID_383 "Offset"; OutVarName_383 "Output Variable"; DataType_DID_384 "DID Monitoring DataType"; ResolDID_384 "Resolution"; OffsetDID_384 "Offset"; OutVarName_384 "Output Variable"; DataType_DID_385 "DID Monitoring DataType"; ResolDID_385 "Resolution"; OffsetDID_385 "Offset"; OutVarName_385 "Output Variable"; DataType_DID_386 "DID Monitoring DataType"; ResolDID_386 "Resolution"; OffsetDID_386 "Offset"; OutVarName_386 "Output Variable"; DataType_DID_387 "DID Monitoring DataType"; ResolDID_387 "Resolution"; OffsetDID_387 "Offset"; OutVarName_387 "Output Variable"; DataType_DID_388 "DID Monitoring DataType"; ResolDID_388 "Resolution"; OffsetDID_388 "Offset"; OutVarName_388 "Output Variable"; DataType_DID_389 "DID Monitoring DataType"; ResolDID_389 "Resolution"; OffsetDID_389 "Offset"; OutVarName_389 "Output Variable"; DataType_DID_390 "DID Monitoring DataType"; ResolDID_390 "Resolution"; OffsetDID_390 "Offset"; OutVarName_390 "Output Variable"; DataType_DID_391 "DID Monitoring DataType"; ResolDID_391 "Resolution"; OffsetDID_391 "Offset"; OutVarName_391 "Output Variable"; DataType_DID_392 "DID Monitoring DataType"; ResolDID_392 "Resolution"; OffsetDID_392 "Offset"; OutVarName_392 "Output Variable"; DataType_DID_393 "DID Monitoring DataType"; ResolDID_393 "Resolution"; OffsetDID_393 "Offset"; OutVarName_393 "Output Variable"; DataType_DID_394 "DID Monitoring DataType"; ResolDID_394 "Resolution"; OffsetDID_394 "Offset"; OutVarName_394 "Output Variable"; DataType_DID_395 "DID Monitoring DataType"; ResolDID_395 "Resolution"; OffsetDID_395 "Offset"; OutVarName_395 "Output Variable"; DataType_DID_396 "DID Monitoring DataType"; ResolDID_396 "Resolution"; OffsetDID_396 "Offset"; OutVarName_396 "Output Variable"; DataType_DID_397 "DID Monitoring DataType"; ResolDID_397 "Resolution"; OffsetDID_397 "Offset"; OutVarName_397 "Output Variable"; DataType_DID_398 "DID Monitoring DataType"; ResolDID_398 "Resolution"; OffsetDID_398 "Offset"; OutVarName_398 "Output Variable"; DataType_DID_399 "DID Monitoring DataType"; ResolDID_399 "Resolution"; OffsetDID_399 "Offset"; OutVarName_399 "Output Variable"; DataType_DID_400 "DID Monitoring DataType"; ResolDID_400 "Resolution"; OffsetDID_400 "Offset"; OutVarName_400 "Output Variable"
      mask help:
      | This function requests the application to write a data value of a DID.
      | Reference to AUTOSAR specification:
      | - AUTOSAR Service Name:  Xxx_WriteData (Ref. [SWS_Dcm_00794])
      |
      | -INPUTS-
      | Generic_Conditions_Write: Generic condition
      | Specific_Conditions_Write_xxxx: Specific condition of DID Variable
      | Configuration Management: Configuration Management (TRUE or FALSE)
      | -PARAMETERS-
      | DID Abstract: Abstract of DID pre-defined
      | Range of DID Variable: 	Range of DID Variable
      | Offset of DID Variable: 	Offset of DID Variable
      | Resolution of DID Variable: 	Resolution of DID Variable
      | Size of DID Variable: 	Byte Number of DID Variable
      | NVM WriteOnFly Variables:  Checked if variables are NVM EEPROM DID variables.
      |
      | Notes: In case where option NVM WriteOnFly Variables is checked. Channel Name should be name of name of specification without prefix and suffix. Example, channel Name should be PTSP_MWIN_GBX_agbtqlimcs.
      mask init:
      | libb= gcb;% get the block name with path
      | libh = get_param(libb,'handle');
      | DIDAbstractstr = get_param(libb,'DIDAbstract');
      | % Callbkstr = strcat('DataServices_',strtrim(DIDAbstractstr),'_WriteData');
      | buff_size = 0;
      | countDID = [];
      | NewStatusstr = '';
      | OldStatusstr = '';
      | count_DID = str2double(get(libh,'NumDIDVar'));
      | conv_subs = [libb,'/Conversion_Subsystem'];
      | data_converter = [libb,'/Data_Type_Conversion'];
      | DMux = [libb,'/Demux'];
      | % wr_fly = [libb,'/AEMS_NVM_WRITEONFLY'];
      | perm_sub = [libb,'/Permission_Subsystem'];
      | old_txtvisibility = get(libh,'AttributesFormatString');
      | %Getting the details for new blocks
      | for i=1:count_DID
      |     n = num2str(i);
      |     
      |     NewStatusstr(i).DID_DataType = get(libh,['DataType_DID_',n]);
      |     NewStatusstr(i).Resol = get(libh,['ResolDID_',n]);
      |     NewStatusstr(i).Offset = get(libh,['OffsetDID_',n]);
      |     NewStatusstr(i).Name = get(libh,['OutVarName_',n]);
      | end
      | 
      | %Getting the details of the old blocks
      | k = find_system(libb,'FollowLinks','on','LookunderMasks','all','regexp','on','Name','^Conversion_Subsystem');
      | ou = {};
      | for i = 1:length(k)
      |     if i==1
      |         conv_blk_name = [libb,'/Conversion_Subsystem'];
      |     else
      |         conv_blk_name = [libb,'/Conversion_Subsystem_',num2str(i)];
      |     end
      |     OldStatusstr(i).DID_DataType = get_param(conv_blk_name,'DID_Datatype');
      |     OldStatusstr(i).Resol = get_param(conv_blk_name,'Resol');
      |     OldStatusstr(i).Offset = get_param(conv_blk_name,'offset');
      |     convertblk=get_param(conv_blk_name,'LineHandles');
      |     dstconvhdl=get_param(convertblk.Outport,'DstBlockHandle');%handle of Data converter block
      |     dstconvlh = get(dstconvhdl,'LineHandles');
      |     dstblkhdl=get_param(dstconvlh.Outport,'DstBlockHandle');%handle of outport
      |     OldStatusstr(i).Name='';
      |     if length(dstblkhdl)==1
      |         OldStatusstr(i).Name=get_param(dstblkhdl,'Name');
      |         ou{end+1} = dstblkhdl;
      |     elseif length(dstblkhdl) > 1
      |         if isequal(get_param(dstblkhdl(1),'BlockType'),'Outport')
      |             OldStatusstr(i).Name=get_param(dstblkhdl(1),'Name');
      |             ou{end+1} = dstblkhdl(1);
      |         elseif isequal(get_param(dstblkhdl(2),'BlockType'),'Outport')
      |             OldStatusstr(i).Name=get_param(dstblkhdl(2),'Name');
      |             ou{end+1} = dstblkhdl(2);
      |         end
      |     end
      | end
      | 
      | chg_status = 0;
      | if length(NewStatusstr) ~= length(OldStatusstr)
      |     chg_status = 1;
      | else %if ~isequal(NewStatusstr,OldStatusstr)
      |     blocks_size=length(NewStatusstr);
      |     if ~isequal({NewStatusstr.DID_DataType},{OldStatusstr.DID_DataType})
      |         chg_status = 1;
      |     end
      | end
      | old_pos_dmux = get_param(DMux,'Position');
      | 
      | if chg_status
      |     lh_dmux = get_param(DMux,'LineHandles');
      |     for a=1:length(lh_dmux.Outport)
      |         try
      |             delete_line(lh_dmux.Outport(a));
      |         catch
      |             %                 disp('unable to delete line');
      |         end
      |     end
      |     dmx_outs = '[';
      |     for i=1:count_DID
      |         if ismember(NewStatusstr(i).DID_DataType,{'uint8','int8'})
      |             This_DID_Size = '1';
      |         elseif ismember(NewStatusstr(i).DID_DataType,{'uint16','int16'})
      |             This_DID_Size = '2';
      |         else%IF the ctrl reaches here means it's uint32 or int32.
      |             This_DID_Size = '4';
      |         end
      |         if i==count_DID
      |             dmx_outs = [dmx_outs,This_DID_Size,']'];
      |         else
      |             dmx_outs = [dmx_outs,This_DID_Size,','];
      |         end
      |     end
      |     % no.of outputs of demux block
      |     set_param(DMux,'Outputs',dmx_outs);
      |     
      |     % dummy values in const block
      |     upd_dmux = get_param(DMux,'PortHandles');
      |     p_upd_dmux = get(upd_dmux.Inport,'Position');
      |     ph_dmux = get_param(DMux,'PortHandles');
      |     
      |     pos_1 = get_param([libb,'/Conversion_Subsystem'],'Position');
      |     Position = old_pos_dmux;
      |     Position(2) = old_pos_dmux(2);
      |     Position(4) = old_pos_dmux(2)+2*20+(pos_1(4)-pos_1(2))*count_DID+(count_DID-1)*60;
      |     set_param(DMux,'Position',Position);
      |     
      |     if length(NewStatusstr) ~= length(OldStatusstr)
      |         if length(NewStatusstr) > length(OldStatusstr)
      |             blocks_size = length(OldStatusstr);
      |             for r=length(OldStatusstr)+1:length(NewStatusstr)
      |                 if r==length(OldStatusstr)+1 && length(OldStatusstr)==1
      |                     pos_r_1 = get_param([libb,'/Conversion_Subsystem'],'Position');
      |                     pos_dc_1 = get_param([libb,'/Data_Type_Conversion'],'Position');
      |                 else
      |                     pos_r_1 = get_param([libb,'/Conversion_Subsystem_',num2str(r-1)],'Position');
      |                     pos_dc_1 = get_param([libb,'/Data_Type_Conversion_',num2str(r-1)],'Position');
      |                 end
      |                 pos_r=pos_r_1;%positions of the new conversion block
      |                 pos_r(2)=pos_r_1(4)+40;
      |                 pos_r(4)=pos_r_1(4)+40+pos_r_1(4)-pos_r_1(2);
      |                 pos_dc=pos_dc_1;%positions of the new data converter block
      |                 pos_dc(2)=pos_dc_1(2)+80;
      |                 pos_dc(4)=pos_dc_1(4)+80;
      |                 if ismember(NewStatusstr(r).DID_DataType,{'uint8','int8'})
      |                     %If the ctrl reaches here means it's a 1 byte
      |                     %input;
      |                     sub_hand = add_block('AEMS_Standard_Library/SUB/AEMS_CONVERT_BYTE_TO_FLP',[libb,'/Conversion_Subsystem_',num2str(r)],'Position',pos_r);
      |                     sub_dc = add_block('simulink/Signal Attributes/Data Type Conversion',[libb,'/Data_Type_Conversion_',num2str(r)],'Position',pos_dc, ...
      |                         'ShowName','off', 'OutDataTypeStr', 'Inherit: Inherit via back propagation');
      |                 else
      |                     sub_hand = add_block('AEMS_Standard_Library/SUB/AEMS_CONVERT_BUFFER_TO_FLP',[libb,'/Conversion_Subsystem_',num2str(r)],'Position',pos_r);
      |                     sub_dc = add_block('simulink/Signal Attributes/Data Type Conversion',[libb,'/Data_Type_Conversion_',num2str(r)],'Position',pos_dc,...
      |                         'ShowName','off', 'OutDataTypeStr', 'Inherit: Inherit via back propagation');
      |                 end
      |                 
      |                 %                 set_param(sub_hand,'Position',pos_r);
      |                 op_hand = add_block('built-in/Outport',[libb,'/',NewStatusstr(r).Name]);
      |                 set_param(op_hand,'Position',[pos_r(1)+400 pos_r(2)+((pos_r(4)-pos_r(2))/2)-7 pos_r(1)+420 pos_r(2)+((pos_r(4)-pos_r(2))/2)+7],'Backgroundcolor','Orange')
      |                 ph_sub = get(sub_hand,'PortHandles');
      |                 ph_dc = get(sub_dc,'PortHandles');
      |                 ph_op = get(op_hand,'PortHandles');
      |                 add_line(libb,ph_sub.Outport,ph_dc.Inport,'Autorouting','On');
      |                 add_line(libb,ph_dc.Outport,ph_op.Inport,'Autorouting','On');
      |             end
      |             
